simulink model "mrefrobotarm_modified_previous_y_previous_u_previous_ref"  (R2018b)
settings: Solver=FixedStepAuto  StartTime=0.0  StopTime=10  RelTol=1e-3  AbsTol=1e-6
undefined symbols (not defined in the file or in its folder): options, sfunxy2
libraries: neural x949, simulink x1
(part 17 of 31)

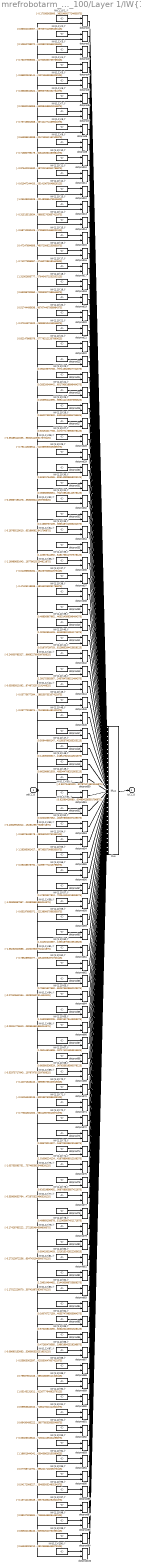
== system mrefrobotarm_modified_previous_y_previous_u_previous_ref/const_51traces_100/Layer 1/IW{1,1} ==
  "pd{1,1}" : Inport  PortDimensions=10
      mask Display: e = 0.06;c1 = [120 230 180]/255;c2 = ([120 230 180]+0)/(256+128);c3 = ([120 230 180]+128)/(256+128);patch([0 1 1 0],[0 0 1 1],c1);patch([0 1 1 1-e 1-e 0+e],[0 0 1 1-e 0+e 0+e],c2);patch([0 0 1 1-e 0+e 0+e],[0 1 1 1-e 1-e 0+e],c3);plot([0 1 1 0 0],[0 0 1 1 0]);
  "IW{1,1}(1,:)'" : Constant  Value=[-0.170305638008138859884610383232939057052135467529296875;-0.84091694602573696659675306364079006016254425048828125;-1.0473111215097110626714993486530147492885589599609375;-0.75666745499568965893644190146005712449550628662109375;0.1371939523011656281159531545199570246040821075439453125;-0.2076176579548360268123730065781273879110813140869140625;0.6369796280798090126751276329741813242435455322265625;0.9908763324366562930123336627730168402194976806640625;1.002178449147427041765467947698198258876800537109375;-0.82460061242790094748755791442818008363246917724609375]
      mask Display: e = 0.06;c1 = [120 150 230]/255;c2 = ([120 150 230]+0)/383;c3 = ([120 150 230]+128)/383;patch([0 1 1 0],[0 0 1 1],c1);patch([0 1 1 1-e 1-e 0+e],[0 0 1 1-e 0+e 0+e],c2);patch([0 0 1 1-e 0+e 0+e],[0 1 1 1-e 1-e 0+e],c3);plot([0 1 1 0 0],[0 0 1 1 0]);disp('Weights');
  "IW{1,1}(10,:)'" : Constant  Value=[-0.7188079917996403889191014968673698604106903076171875;-0.5527934950988353524081730938632972538471221923828125;1.177940059427081909149137572967447340488433837890625;-0.7566037792006319318005580498720519244670867919921875;0.10224905637283122905589749507271335460245609283447265625;0.880612868538781068394882822758518159389495849609375;0.05599996081731146990723146927848574705421924591064453125;-0.5350580343929980386974420980550348758697509765625;-0.73962591974704261499340418595238588750362396240234375;-0.01401764490016039164943517647543558268807828426361083984375]
      mask Display: e = 0.06;c1 = [120 150 230]/255;c2 = ([120 150 230]+0)/383;c3 = ([120 150 230]+128)/383;patch([0 1 1 0],[0 0 1 1],c1);patch([0 1 1 1-e 1-e 0+e],[0 0 1 1-e 0+e 0+e],c2);patch([0 0 1 1-e 0+e 0+e],[0 1 1 1-e 1-e 0+e],c3);plot([0 1 1 0 0],[0 0 1 1 0]);disp('Weights');
  "IW{1,1}(100,:)'" : Constant  Value=[0.64533025212050676433506168905296362936496734619140625;0.8803140978111179126841534525738097727298736572265625;0.54439970602968112967090519305202178657054901123046875;-0.53792355137469483050693952463916502892971038818359375;-1.2233752874797414467167300244909711182117462158203125;-0.375810009441459980106259308740845881402492523193359375;0.40564792046065389907738563124439679086208343505859375;0.542278062316380538021576285245828330516815185546875;0.338638468446645746201539850517292506992816925048828125;-0.05135870021747131197731306428977404721081256866455078125]
      mask Display: e = 0.06;c1 = [120 150 230]/255;c2 = ([120 150 230]+0)/383;c3 = ([120 150 230]+128)/383;patch([0 1 1 0],[0 0 1 1],c1);patch([0 1 1 1-e 1-e 0+e],[0 0 1 1-e 0+e 0+e],c2);patch([0 0 1 1-e 0+e 0+e],[0 1 1 1-e 1-e 0+e],c3);plot([0 1 1 0 0],[0 0 1 1 0]);disp('Weights');
  "IW{1,1}(11,:)'" : Constant  Value=[-0.97642024630729606915480189854861237108707427978515625;0.66445209408851069188273186227888800203800201416015625;-0.8919160165742419099643711888347752392292022705078125;0.10756129521181546915276072695633047260344028472900390625;-0.6447824446878331894339453356224112212657928466796875;0.67602283036553612038943583684158511459827423095703125;1.0285614969354053283012717656674794852733612060546875;-0.77894280059782949887647873765672557055950164794921875;-0.1748333285319037810889852835316560231149196624755859375;-0.41474870595583002153006191292661242187023162841796875]
      mask Display: e = 0.06;c1 = [120 150 230]/255;c2 = ([120 150 230]+0)/383;c3 = ([120 150 230]+128)/383;patch([0 1 1 0],[0 0 1 1],c1);patch([0 1 1 1-e 1-e 0+e],[0 0 1 1-e 0+e 0+e],c2);patch([0 0 1 1-e 0+e 0+e],[0 1 1 1-e 1-e 0+e],c3);plot([0 1 1 0 0],[0 0 1 1 0]);disp('Weights');
  "IW{1,1}(12,:)'" : Constant  Value=[-0.6194724442048145096606504012015648186206817626953125;-0.72861833503561956870697713384288363158702850341796875;1.103333456587284100436363587505184113979339599609375;-0.70243798980666405373796123967622406780719757080078125;0.439153999977970499468682419319520704448223114013671875;0.45345915572852302233286536647938191890716552734375;-0.34918842111248615811547324483399279415607452392578125;-0.8964166863968896503678251974633894860744476318359375;-0.43450253988920584102828570394194684922695159912109375;0.1004094661472918759148598155661602504551410675048828125]
      mask Display: e = 0.06;c1 = [120 150 230]/255;c2 = ([120 150 230]+0)/383;c3 = ([120 150 230]+128)/383;patch([0 1 1 0],[0 0 1 1],c1);patch([0 1 1 1-e 1-e 0+e],[0 0 1 1-e 0+e 0+e],c2);patch([0 0 1 1-e 0+e 0+e],[0 1 1 1-e 1-e 0+e],c3);plot([0 1 1 0 0],[0 0 1 1 0]);disp('Weights');
  "IW{1,1}(13,:)'" : Constant  Value=[1.25349304526054883268670891993679106235504150390625;-0.278560517477228819505086221397505141794681549072265625;0.730108871976856477203909889794886112213134765625;-0.549904814972676181383803850621916353702545166015625;0.62399252602846766446731407995685003697872161865234375;-1.281837938187930792111046685022301971912384033203125;0.345251730969751757793773094817879609763622283935546875;0.138568870452370263013364137805183418095111846923828125;-0.58106563584299875113714506369433365762233734130859375;-0.36006533748797819871612091446877457201480865478515625]
      mask Display: e = 0.06;c1 = [120 150 230]/255;c2 = ([120 150 230]+0)/383;c3 = ([120 150 230]+128)/383;patch([0 1 1 0],[0 0 1 1],c1);patch([0 1 1 1-e 1-e 0+e],[0 0 1 1-e 0+e 0+e],c2);patch([0 0 1 1-e 0+e 0+e],[0 1 1 1-e 1-e 0+e],c3);plot([0 1 1 0 0],[0 0 1 1 0]);disp('Weights');
  "IW{1,1}(14,:)'" : Constant  Value=[-0.3151351363461738497306896533700637519359588623046875;-0.0097595836595271122371197947131804539822041988372802734375;1.10936805191082843435879112803377211093902587890625;-0.93905292104770021754944764325045980513095855712890625;-0.9138700935437042982556476999889127910137176513671875;0.18374239433762584727816147278645075857639312744140625;1.069462447122071946381538509740494191646575927734375;-0.81828312627598853712385107428417541086673736572265625;-0.023265579288859618289908581800773390568792819976806640625;0.1571687035658450859454404735515709035098552703857421875]
      mask Display: e = 0.06;c1 = [120 150 230]/255;c2 = ([120 150 230]+0)/383;c3 = ([120 150 230]+128)/383;patch([0 1 1 0],[0 0 1 1],c1);patch([0 1 1 1-e 1-e 0+e],[0 0 1 1-e 0+e 0+e],c2);patch([0 0 1 1-e 0+e 0+e],[0 1 1 1-e 1-e 0+e],c3);plot([0 1 1 0 0],[0 0 1 1 0]);disp('Weights');
  "IW{1,1}(15,:)'" : Constant  Value=[-0.5871293042540719486765965484664775431156158447265625;0.3940422689418039414732675140840001404285430908203125;0.96312911671125911450275225433870218694210052490234375;-1.01431590084022449360645623528398573398590087890625;-0.325931841206041406078242061994387768208980560302734375;0.200414918554812360174111063315649516880512237548828125;0.331194186191319073220284963099402375519275665283203125;1.2119257407114261138048050270299427211284637451171875;-0.8267099033237830241205301717855036258697509765625;0.10958005298265061089324490239960141479969024658203125]
      mask Display: e = 0.06;c1 = [120 150 230]/255;c2 = ([120 150 230]+0)/383;c3 = ([120 150 230]+128)/383;patch([0 1 1 0],[0 0 1 1],c1);patch([0 1 1 1-e 1-e 0+e],[0 0 1 1-e 0+e 0+e],c2);patch([0 0 1 1-e 0+e 0+e],[0 1 1 1-e 1-e 0+e],c3);plot([0 1 1 0 0],[0 0 1 1 0]);disp('Weights');
  "IW{1,1}(16,:)'" : Constant  Value=[0.472476948566088517100780563851003535091876983642578125;0.436399456262539231499175684803049080073833465576171875;1.0138022013108933805369815672747790813446044921875;-0.825843001599289916470070238574407994747161865234375;0.239318836898521347666957126421038992702960968017578125;-0.6405951194830503681032496388070285320281982421875;-0.71669483108157117090541987636242993175983428955078125;-0.5155833539305538781860605013207532465457916259765625;0.320021634560399836910704607362276874482631683349609375;1.1416495802142418991564909447333775460720062255859375]
      mask Display: e = 0.06;c1 = [120 150 230]/255;c2 = ([120 150 230]+0)/383;c3 = ([120 150 230]+128)/383;patch([0 1 1 0],[0 0 1 1],c1);patch([0 1 1 1-e 1-e 0+e],[0 0 1 1-e 0+e 0+e],c2);patch([0 0 1 1-e 0+e 0+e],[0 1 1 1-e 1-e 0+e],c3);plot([0 1 1 0 0],[0 0 1 1 0]);disp('Weights');
  "IW{1,1}(17,:)'" : Constant  Value=[-0.74077896967243128667490736916079185903072357177734375;-0.2975123869242335405971289219451136887073516845703125;0.39331342274744585107981720284442417323589324951171875;-0.12030082952774480420377045675195404328405857086181640625;0.97014414268526094620170852067531086504459381103515625;-0.8509573298599459878488460162770934402942657470703125;-0.82800102302075317961538303279667161405086517333984375;0.86967158602187566440733235140214674174785614013671875;-0.314482355644385702664322934651863761246204376220703125;0.42603053129348611438587113298126496374607086181640625]
      mask Display: e = 0.06;c1 = [120 150 230]/255;c2 = ([120 150 230]+0)/383;c3 = ([120 150 230]+128)/383;patch([0 1 1 0],[0 0 1 1],c1);patch([0 1 1 1-e 1-e 0+e],[0 0 1 1-e 0+e 0+e],c2);patch([0 0 1 1-e 0+e 0+e],[0 1 1 1-e 1-e 0+e],c3);plot([0 1 1 0 0],[0 0 1 1 0]);disp('Weights');
  "IW{1,1}(18,:)'" : Constant  Value=[1.3100269377766393663620192455709911882877349853515625;-0.57664102931916350058827447355724871158599853515625;0.326570474994216708441996388501138426363468170166015625;-0.307961676870106060288634353128145448863506317138671875;0.82859508544864846069089026059373281896114349365234375;1.160795476552283655991004707175306975841522216796875;-0.0156597094076652391947401810057272086851298809051513671875;-0.350765766554864522053236441934132017195224761962890625;-0.058250586835098878968342006601233151741325855255126953125;-0.81675852122060366156119926017709076404571533203125]
      mask Display: e = 0.06;c1 = [120 150 230]/255;c2 = ([120 150 230]+0)/383;c3 = ([120 150 230]+128)/383;patch([0 1 1 0],[0 0 1 1],c1);patch([0 1 1 1-e 1-e 0+e],[0 0 1 1-e 0+e 0+e],c2);patch([0 0 1 1-e 0+e 0+e],[0 1 1 1-e 1-e 0+e],c3);plot([0 1 1 0 0],[0 0 1 1 0]);disp('Weights');
  "IW{1,1}(19,:)'" : Constant  Value=[0.632867829608980247968474941444583237171173095703125;-0.0743945784967924572672615113333449698984622955322265625;-0.91327949984337830624525622624787501990795135498046875;-0.82963064081226456369932975576375611126422882080078125;0.46425932832785410386833291340735740959644317626953125;0.462075831172123641099602764370501972734928131103515625;-0.4812285572585504045406423756503500044345855712890625;-0.01180364781508570770629518165151239372789859771728515625;-1.21000651010020288111945774289779365062713623046875;-1.0575192814166551880106226235511712729930877685546875]
      mask Display: e = 0.06;c1 = [120 150 230]/255;c2 = ([120 150 230]+0)/383;c3 = ([120 150 230]+128)/383;patch([0 1 1 0],[0 0 1 1],c1);patch([0 1 1 1-e 1-e 0+e],[0 0 1 1-e 0+e 0+e],c2);patch([0 0 1 1-e 0+e 0+e],[0 1 1 1-e 1-e 0+e],c3);plot([0 1 1 0 0],[0 0 1 1 0]);disp('Weights');
  "IW{1,1}(2,:)'" : Constant  Value=[0.86302163357631755946641760601778514683246612548828125;-0.5579812505175449910410634402069263160228729248046875;-0.8557487905362055613522898056544363498687744140625;-0.514363216250348642688550171442329883575439453125;-0.975544136415781082405374036170542240142822265625;0.4210426174550914169003590359352529048919677734375;-0.63869385442526571683430347547982819378376007080078125;0.65062821069079068703189250300056301057338714599609375;0.35157843060015958602804175825440324842929840087890625;0.86647648865104731630282230980810709297657012939453125]
      mask Display: e = 0.06;c1 = [120 150 230]/255;c2 = ([120 150 230]+0)/383;c3 = ([120 150 230]+128)/383;patch([0 1 1 0],[0 0 1 1],c1);patch([0 1 1 1-e 1-e 0+e],[0 0 1 1-e 0+e 0+e],c2);patch([0 0 1 1-e 0+e 0+e],[0 1 1 1-e 1-e 0+e],c3);plot([0 1 1 0 0],[0 0 1 1 0]);disp('Weights');
  "IW{1,1}(20,:)'" : Constant  Value=[0.51744495636959675355370791294262744486331939697265625;-0.1547734165125060623591224384654196910560131072998046875;-0.99093210573097934013020449128816835582256317138671875;0.263933305768935422275234259359422139823436737060546875;-0.0728289172390254313516066986267105676233768463134765625;-0.47621939097836063492508174022077582776546478271484375;-1.1292248128611817037381115369498729705810546875;-0.041618293867331478119719889718908234499394893646240234375;-1.0841222482710100027958333157585002481937408447265625;0.189330866318472512688231290667317807674407958984375]
      mask Display: e = 0.06;c1 = [120 150 230]/255;c2 = ([120 150 230]+0)/383;c3 = ([120 150 230]+128)/383;patch([0 1 1 0],[0 0 1 1],c1);patch([0 1 1 1-e 1-e 0+e],[0 0 1 1-e 0+e 0+e],c2);patch([0 0 1 1-e 0+e 0+e],[0 1 1 1-e 1-e 0+e],c3);plot([0 1 1 0 0],[0 0 1 1 0]);disp('Weights');
  "IW{1,1}(21,:)'" : Constant  Value=[-0.371518715204130212104161046227090992033481597900390625;0.467337757155769306649517602636478841304779052734375;0.2269719081821011397170906320752692408859729766845703125;0.08481228167460937161781231452550855465233325958251953125;1.44458428183304032899059166084043681621551513671875;-0.0234380543474412873783396804583389894105494022369384765625;-0.45455741294511387007304392682272009551525115966796875;-1.227396331157477593620797051698900759220123291015625;1.004787797655553038822517919470556080341339111328125;0.1506891507751337566656246735874447040259838104248046875]
      mask Display: e = 0.06;c1 = [120 150 230]/255;c2 = ([120 150 230]+0)/383;c3 = ([120 150 230]+128)/383;patch([0 1 1 0],[0 0 1 1],c1);patch([0 1 1 1-e 1-e 0+e],[0 0 1 1-e 0+e 0+e],c2);patch([0 0 1 1-e 0+e 0+e],[0 1 1 1-e 1-e 0+e],c3);plot([0 1 1 0 0],[0 0 1 1 0]);disp('Weights');
  "IW{1,1}(22,:)'" : Constant  Value=[0.8214786607933863837871513169375248253345489501953125;-0.84220472360854403692798086922266520559787750244140625;-0.4880387325338571002930621034465730190277099609375;0.60696914376156396730976894104969687759876251220703125;-0.887166316198694016037507026339881122112274169921875;0.79926168947075215687192439872887916862964630126953125;0.80816360662084540944505306470091454684734344482421875;-0.5721497555960544101338882683194242417812347412109375;0.567110586128520832716048971633426845073699951171875;0.460100559308461110052945741699659265577793121337890625]
      mask Display: e = 0.06;c1 = [120 150 230]/255;c2 = ([120 150 230]+0)/383;c3 = ([120 150 230]+128)/383;patch([0 1 1 0],[0 0 1 1],c1);patch([0 1 1 1-e 1-e 0+e],[0 0 1 1-e 0+e 0+e],c2);patch([0 0 1 1-e 0+e 0+e],[0 1 1 1-e 1-e 0+e],c3);plot([0 1 1 0 0],[0 0 1 1 0]);disp('Weights');
  "IW{1,1}(23,:)'" : Constant  Value=[0.09419575738046971624672920597731717862188816070556640625;0.411730692981060186763642150253872387111186981201171875;0.41947599709186744743050212491652928292751312255859375;-0.51148504298385499833301537364604882895946502685546875;-0.70916810981691391635450827379827387630939483642578125;-1.16257670448549976782715020817704498767852783203125;-0.9791973104793552096225539571605622768402099609375;1.0943516112241928883719310761080123484134674072265625;0.3134970998681072540392733571934513747692108154296875;0.379077417386230075546649231910123489797115325927734375]
      mask Display: e = 0.06;c1 = [120 150 230]/255;c2 = ([120 150 230]+0)/383;c3 = ([120 150 230]+128)/383;patch([0 1 1 0],[0 0 1 1],c1);patch([0 1 1 1-e 1-e 0+e],[0 0 1 1-e 0+e 0+e],c2);patch([0 0 1 1-e 0+e 0+e],[0 1 1 1-e 1-e 0+e],c3);plot([0 1 1 0 0],[0 0 1 1 0]);disp('Weights');
  "IW{1,1}(24,:)'" : Constant  Value=[0.283200494423681170541584606326068751513957977294921875;-0.5446401217881791101405042354599572718143463134765625;-0.926718550507767968582584217074327170848846435546875;1.0023171860421360435111637343652546405792236328125;-0.401982680773332823331855934156919829547405242919921875;0.255525526075908226975030856920056976377964019775390625;0.89032793712451674394969813874922692775726318359375;1.0527621924029799682642760672024451196193695068359375;-0.36601162666097974973666850928566418588161468505859375;-0.6552325421269118432832101461826823651790618896484375]
      mask Display: e = 0.06;c1 = [120 150 230]/255;c2 = ([120 150 230]+0)/383;c3 = ([120 150 230]+128)/383;patch([0 1 1 0],[0 0 1 1],c1);patch([0 1 1 1-e 1-e 0+e],[0 0 1 1-e 0+e 0+e],c2);patch([0 0 1 1-e 0+e 0+e],[0 1 1 1-e 1-e 0+e],c3);plot([0 1 1 0 0],[0 0 1 1 0]);disp('Weights');
  "IW{1,1}(25,:)'" : Constant  Value=[0.263952423958710491458390379193588159978389739990234375;0.5179072584720512129052849559229798614978790283203125;-0.07410029705099137331547609619519789703190326690673828125;-0.871104755366767680158091025077737867832183837890625;-0.903016070580165308712139449198730289936065673828125;0.7666990005644398475936895920312963426113128662109375;-0.8009951831969763791363448035554029047489166259765625;0.2222925408359026910876110605386202223598957061767578125;0.925174136198293250998858638922683894634246826171875;-0.86957339748055384465175166042172349989414215087890625]
      mask Display: e = 0.06;c1 = [120 150 230]/255;c2 = ([120 150 230]+0)/383;c3 = ([120 150 230]+128)/383;patch([0 1 1 0],[0 0 1 1],c1);patch([0 1 1 1-e 1-e 0+e],[0 0 1 1-e 0+e 0+e],c2);patch([0 0 1 1-e 0+e 0+e],[0 1 1 1-e 1-e 0+e],c3);plot([0 1 1 0 0],[0 0 1 1 0]);disp('Weights');
  "IW{1,1}(26,:)'" : Constant  Value=[0.66207392930839847888790927754598669707775115966796875;-0.927826293094271559169783358811400830745697021484375;-0.53992479788772340665303772766492329537868499755859375;0.6093454934288307089929048743215389549732208251953125;-0.935697886848097848400129805668257176876068115234375;0.1275534011237173526165378234509262256324291229248046875;-0.71002476471670294966287428906070999801158905029296875;-0.6154051848111132816399049261235632002353668212890625;1.1040911523030134677725300207384862005710601806640625;-0.006260111974622986109884070771158803836442530155181884765625]
      mask Display: e = 0.06;c1 = [120 150 230]/255;c2 = ([120 150 230]+0)/383;c3 = ([120 150 230]+128)/383;patch([0 1 1 0],[0 0 1 1],c1);patch([0 1 1 1-e 1-e 0+e],[0 0 1 1-e 0+e 0+e],c2);patch([0 0 1 1-e 0+e 0+e],[0 1 1 1-e 1-e 0+e],c3);plot([0 1 1 0 0],[0 0 1 1 0]);disp('Weights');
  "IW{1,1}(27,:)'" : Constant  Value=[0.6319401773805248812010404435568489134311676025390625;-0.84957682223790575992694584783748723566532135009765625;0.5357136767300738622310518621816299855709075927734375;-0.88565078629698656964563951987656764686107635498046875;-1.0552096523122538318517626976245082914829254150390625;0.88306545275100223335584814776666462421417236328125;0.826385453474836051412921733572147786617279052734375;0.046199217615886183085915916990416008047759532928466796875;-0.2139731479252826584769309192779473960399627685546875;0.07682384842362673105231607451059971936047077178955078125]
      mask Display: e = 0.06;c1 = [120 150 230]/255;c2 = ([120 150 230]+0)/383;c3 = ([120 150 230]+128)/383;patch([0 1 1 0],[0 0 1 1],c1);patch([0 1 1 1-e 1-e 0+e],[0 0 1 1-e 0+e 0+e],c2);patch([0 0 1 1-e 0+e 0+e],[0 1 1 1-e 1-e 0+e],c3);plot([0 1 1 0 0],[0 0 1 1 0]);disp('Weights');
  "IW{1,1}(28,:)'" : Constant  Value=[-0.39489441535742753064397447815281338989734649658203125;0.047164668367843463891997402015476836822926998138427734375;0.73428078885034953060539919533766806125640869140625;-0.5170768242902992195553224519244395196437835693359375;-0.650913494200199949091256712563335895538330078125;-0.29069613486833978388546029236749745905399322509765625;0.685236331361608108636573888361454010009765625;1.4916971807746828293517182828509248793125152587890625;0.8581651008094379751156566271674819290637969970703125;-0.0231304909361202577777749667120588128454983234405517578125]
      mask Display: e = 0.06;c1 = [120 150 230]/255;c2 = ([120 150 230]+0)/383;c3 = ([120 150 230]+128)/383;patch([0 1 1 0],[0 0 1 1],c1);patch([0 1 1 1-e 1-e 0+e],[0 0 1 1-e 0+e 0+e],c2);patch([0 0 1 1-e 0+e 0+e],[0 1 1 1-e 1-e 0+e],c3);plot([0 1 1 0 0],[0 0 1 1 0]);disp('Weights');
  "IW{1,1}(29,:)'" : Constant  Value=[-0.791116069143575462163653355673886835575103759765625;-0.5164163335247102804004271092708222568035125732421875;1.134330783552872201624950321274809539318084716796875;-0.50120208438853131038825949872261844575405120849609375;1.31633127280354500499015557579696178436279296875;-0.266539812518394481077876889685285277664661407470703125;-1.1946739896386346924117560774902813136577606201171875;-0.87808470016394990498298511738539673388004302978515625;0.55821663455198378134269887596019543707370758056640625;-0.49625539141540497833915424052975140511989593505859375]
      mask Display: e = 0.06;c1 = [120 150 230]/255;c2 = ([120 150 230]+0)/383;c3 = ([120 150 230]+128)/383;patch([0 1 1 0],[0 0 1 1],c1);patch([0 1 1 1-e 1-e 0+e],[0 0 1 1-e 0+e 0+e],c2);patch([0 0 1 1-e 0+e 0+e],[0 1 1 1-e 1-e 0+e],c3);plot([0 1 1 0 0],[0 0 1 1 0]);disp('Weights');
  "IW{1,1}(3,:)'" : Constant  Value=[0.10552788972297309777470530889331712387502193450927734375;0.88774397676408056678809543882380239665508270263671875;-0.290424624436791900539134303471655584871768951416015625;-0.55515280106611630817070590637740679085254669189453125;0.2495591789322011144758306500079925172030925750732421875;0.518666085829210476987327638198621571063995361328125;-0.7146768557075773298237209019134752452373504638671875;-1.1663537558078445055542715635965578258037567138671875;-0.8429764640291583788211937644518911838531494140625;-0.9813004957389550586555060363025404512882232666015625]
      mask Display: e = 0.06;c1 = [120 150 230]/255;c2 = ([120 150 230]+0)/383;c3 = ([120 150 230]+128)/383;patch([0 1 1 0],[0 0 1 1],c1);patch([0 1 1 1-e 1-e 0+e],[0 0 1 1-e 0+e 0+e],c2);patch([0 0 1 1-e 0+e 0+e],[0 1 1 1-e 1-e 0+e],c3);plot([0 1 1 0 0],[0 0 1 1 0]);disp('Weights');
  "IW{1,1}(30,:)'" : Constant  Value=[0.626017640653714568799159678746946156024932861328125;0.1479782944948506429039269960412639193236827850341796875;0.1393829123997244734400879906388581730425357818603515625;-0.466620041588095502138600068064988590776920318603515625;0.66086884231012976709251915963250212371349334716796875;-0.471986669595617691630451417950098402798175811767578125;-0.2210552926631040027150021387569722719490528106689453125;-1.1080786045275470286242125439457595348358154296875;0.834856584082876107544279875583015382289886474609375;-1.1414665398944816576687344422680325806140899658203125]
      mask Display: e = 0.06;c1 = [120 150 230]/255;c2 = ([120 150 230]+0)/383;c3 = ([120 150 230]+128)/383;patch([0 1 1 0],[0 0 1 1],c1);patch([0 1 1 1-e 1-e 0+e],[0 0 1 1-e 0+e 0+e],c2);patch([0 0 1 1-e 0+e 0+e],[0 1 1 1-e 1-e 0+e],c3);plot([0 1 1 0 0],[0 0 1 1 0]);disp('Weights');
  "IW{1,1}(31,:)'" : Constant  Value=[0.06668568061349466891130077783600427210330963134765625;0.88698937972517466477029302041046321392059326171875;-0.5020620907164901058905570607748813927173614501953125;0.187274332582882896414133711004978977143764495849609375;0.88575747583989616895649987782235257327556610107421875;-0.81825415593434147609741557971574366092681884765625;0.68899848459867774064235845798975788056850433349609375;0.94305114029854142376763093125191517174243927001953125;-0.6691163549777299213161541047156788408756256103515625;0.0737283603405594067936590363387949764728546142578125]
      mask Display: e = 0.06;c1 = [120 150 230]/255;c2 = ([120 150 230]+0)/383;c3 = ([120 150 230]+128)/383;patch([0 1 1 0],[0 0 1 1],c1);patch([0 1 1 1-e 1-e 0+e],[0 0 1 1-e 0+e 0+e],c2);patch([0 0 1 1-e 0+e 0+e],[0 1 1 1-e 1-e 0+e],c3);plot([0 1 1 0 0],[0 0 1 1 0]);disp('Weights');
  "IW{1,1}(32,:)'" : Constant  Value=[-0.29867193478553277774523166954168118536472320556640625;1.060980638567496026070102743688039481639862060546875;-0.83983801109680944474433772484189830720424652099609375;0.287629578909353422755401652466389350593090057373046875;0.51783125481217850971660254799644462764263153076171875;0.283346881376406456443106662845821119844913482666015625;-0.9786366480410244594878577117924578487873077392578125;-1.067149516731294323079737296211533248424530029296875;0.2003698181893468766023858051994466222822666168212890625;-0.67592741568701220078452251982525922358036041259765625]
      mask Display: e = 0.06;c1 = [120 150 230]/255;c2 = ([120 150 230]+0)/383;c3 = ([120 150 230]+128)/383;patch([0 1 1 0],[0 0 1 1],c1);patch([0 1 1 1-e 1-e 0+e],[0 0 1 1-e 0+e 0+e],c2);patch([0 0 1 1-e 0+e 0+e],[0 1 1 1-e 1-e 0+e],c3);plot([0 1 1 0 0],[0 0 1 1 0]);disp('Weights');
  "IW{1,1}(33,:)'" : Constant  Value=[0.116887874095150390285624553143861703574657440185546875;0.63308229908039714839418365954770706593990325927734375;-0.0777111172460257793037641249611624516546726226806640625;-0.78538148508143701409522918766015209257602691650390625;-0.99080372460652810229220222026924602687358856201171875;1.1750499935507499049691659820382483303546905517578125;-0.50299687336723286623652029447839595377445220947265625;-0.2186709169920443007750776587272412143647670745849609375;1.1043639607425597137790873603080399334430694580078125;-0.33939116012177217296397202517255209386348724365234375]
      mask Display: e = 0.06;c1 = [120 150 230]/255;c2 = ([120 150 230]+0)/383;c3 = ([120 150 230]+128)/383;patch([0 1 1 0],[0 0 1 1],c1);patch([0 1 1 1-e 1-e 0+e],[0 0 1 1-e 0+e 0+e],c2);patch([0 0 1 1-e 0+e 0+e],[0 1 1 1-e 1-e 0+e],c3);plot([0 1 1 0 0],[0 0 1 1 0]);disp('Weights');
  "IW{1,1}(34,:)'" : Constant  Value=[-0.187692190106364675816763565308065153658390045166015625;1.2964434572948750901133507795748300850391387939453125;-0.46176563770852829815538598268176428973674774169921875;-0.27552557411780764784481334572774358093738555908203125;-0.603843694195803859514626310556195676326751708984375;-0.5983048122454321937624399652122519910335540771484375;-0.7669376889578789491253019150462932884693145751953125;0.1629662413332511883279352105091675184667110443115234375;0.324312279636630729218182978002005256712436676025390625;-0.20198865888583827921110014358418993651866912841796875]
      mask Display: e = 0.06;c1 = [120 150 230]/255;c2 = ([120 150 230]+0)/383;c3 = ([120 150 230]+128)/383;patch([0 1 1 0],[0 0 1 1],c1);patch([0 1 1 1-e 1-e 0+e],[0 0 1 1-e 0+e 0+e],c2);patch([0 0 1 1-e 0+e 0+e],[0 1 1 1-e 1-e 0+e],c3);plot([0 1 1 0 0],[0 0 1 1 0]);disp('Weights');
  "IW{1,1}(35,:)'" : Constant  Value=[1.2256734439276437687027510037296451628208160400390625;-0.9330947970269434232903904558042995631694793701171875;0.131230327499476773223108239108114503324031829833984375;-0.6805497732182999026662173491786234080791473388671875;0.62001055341251010144532074264134280383586883544921875;0.6535912239619818819846841506659984588623046875;0.62055220915618836130533964023925364017486572265625;0.358587438438109640248541154505801387131214141845703125;-0.61424990739872475931093731560395099222660064697265625;-0.6624892400696531513659692791406996548175811767578125]
      mask Display: e = 0.06;c1 = [120 150 230]/255;c2 = ([120 150 230]+0)/383;c3 = ([120 150 230]+128)/383;patch([0 1 1 0],[0 0 1 1],c1);patch([0 1 1 1-e 1-e 0+e],[0 0 1 1-e 0+e 0+e],c2);patch([0 0 1 1-e 0+e 0+e],[0 1 1 1-e 1-e 0+e],c3);plot([0 1 1 0 0],[0 0 1 1 0]);disp('Weights');
  "IW{1,1}(36,:)'" : Constant  Value=[-1.1698983164396683509522745225694961845874786376953125;0.039703620286117603799258546359851607121527194976806640625;0.07486672289221334153364040275846491567790508270263671875;0.9785601315053107374097862702910788357257843017578125;0.980185417500065714335732991457916796207427978515625;-0.66657049432687376366857279208488762378692626953125;0.5239409712108564765031815113616175949573516845703125;-0.2496624487829249561254840727997361682355403900146484375;-0.86867630952089813778371762964525260031223297119140625;-0.370817217133690923969169261908973567187786102294921875]
      mask Display: e = 0.06;c1 = [120 150 230]/255;c2 = ([120 150 230]+0)/383;c3 = ([120 150 230]+128)/383;patch([0 1 1 0],[0 0 1 1],c1);patch([0 1 1 1-e 1-e 0+e],[0 0 1 1-e 0+e 0+e],c2);patch([0 0 1 1-e 0+e 0+e],[0 1 1 1-e 1-e 0+e],c3);plot([0 1 1 0 0],[0 0 1 1 0]);disp('Weights');
  "IW{1,1}(37,:)'" : Constant  Value=[-0.0149666328452099338386371840670108213089406490325927734375;-0.931936877760145332416641394956968724727630615234375;-1.151949433050794002753036693320609629154205322265625;0.86870508548147118421667300935951061546802520751953125;0.187403977636498686454302742276922799646854400634765625;1.008057905890814343052852564142085611820220947265625;0.092644828769221698738789427807205356657505035400390625;-0.73461588425985924200034560271888040006160736083984375;0.5612002737993935230775832678773440420627593994140625;-0.10958425546422807805857502216895227320492267608642578125]
      mask Display: e = 0.06;c1 = [120 150 230]/255;c2 = ([120 150 230]+0)/383;c3 = ([120 150 230]+128)/383;patch([0 1 1 0],[0 0 1 1],c1);patch([0 1 1 1-e 1-e 0+e],[0 0 1 1-e 0+e 0+e],c2);patch([0 0 1 1-e 0+e 0+e],[0 1 1 1-e 1-e 0+e],c3);plot([0 1 1 0 0],[0 0 1 1 0]);disp('Weights');
  "IW{1,1}(38,:)'" : Constant  Value=[-0.474251185983347089969441867651767097413539886474609375;0.66920382643324760607583812088705599308013916015625;0.64710109619507372169522341209813021123409271240234375;-0.51139914103564210190455696647404693067073822021484375;-0.63816283216853098014809120286372490227222442626953125;0.29697077566583074403894215720356442034244537353515625;-0.71411559907816102299449312340584583580493927001953125;-0.340996826896414029217652341685607098042964935302734375;-1.3192546636798339054763573585660196840763092041015625;-0.83402969627138634489682544881361536681652069091796875]
      mask Display: e = 0.06;c1 = [120 150 230]/255;c2 = ([120 150 230]+0)/383;c3 = ([120 150 230]+128)/383;patch([0 1 1 0],[0 0 1 1],c1);patch([0 1 1 1-e 1-e 0+e],[0 0 1 1-e 0+e 0+e],c2);patch([0 0 1 1-e 0+e 0+e],[0 1 1 1-e 1-e 0+e],c3);plot([0 1 1 0 0],[0 0 1 1 0]);disp('Weights');
  "IW{1,1}(39,:)'" : Constant  Value=[0.4885696796264940022780365325161255896091461181640625;1.0011953446721630900384525375557132065296173095703125;-0.07965199188943576646959598974717664532363414764404296875;-0.14133535981193434682978704586275853216648101806640625;0.7405218790532515082958298080484382808208465576171875;-0.08748518407597898061123231627789209596812725067138671875;-0.13676008771209080538966418316704221069812774658203125;-0.97328788404739630113482462547835893929004669189453125;1.4107007557266684205643514360417611896991729736328125;0.035579408801526289651828705018488108180463314056396484375]
      mask Display: e = 0.06;c1 = [120 150 230]/255;c2 = ([120 150 230]+0)/383;c3 = ([120 150 230]+128)/383;patch([0 1 1 0],[0 0 1 1],c1);patch([0 1 1 1-e 1-e 0+e],[0 0 1 1-e 0+e 0+e],c2);patch([0 0 1 1-e 0+e 0+e],[0 1 1 1-e 1-e 0+e],c3);plot([0 1 1 0 0],[0 0 1 1 0]);disp('Weights');
  "IW{1,1}(4,:)'" : Constant  Value=[-0.76197969360801354188339473694213666021823883056640625;-0.26771973179288444111278977288748137652873992919921875;0.697379882929172634220549298333935439586639404296875;0.1355540479345000992594805211410857737064361572265625;0.52410901792617270444907262572087347507476806640625;-1.0158318151387122352247160961269401013851165771484375;0.8255710489851839639641184476204216480255126953125;-0.99875358677146852670603038859553635120391845703125;-0.71022033136298012845344373999978415668010711669921875;-0.706952677093088510673624114133417606353759765625]
      mask Display: e = 0.06;c1 = [120 150 230]/255;c2 = ([120 150 230]+0)/383;c3 = ([120 150 230]+128)/383;patch([0 1 1 0],[0 0 1 1],c1);patch([0 1 1 1-e 1-e 0+e],[0 0 1 1-e 0+e 0+e],c2);patch([0 0 1 1-e 0+e 0+e],[0 1 1 1-e 1-e 0+e],c3);plot([0 1 1 0 0],[0 0 1 1 0]);disp('Weights');
  "IW{1,1}(40,:)'" : Constant  Value=[1.022626944269706683598997187800705432891845703125;0.09685762306828386847268319570503081195056438446044921875;-0.64434950537638535639217707284842617809772491455078125;0.658483519736270839217695538536645472049713134765625;0.2395668410857852703710335617870441637933254241943359375;0.07937716463412373968377977462296257726848125457763671875;-1.009659204805799515014541611890308558940887451171875;1.149825552452031995898096283781342208385467529296875;-0.456427362312665729771055111996247433125972747802734375;0.52825004028654276577725568131427280604839324951171875]
      mask Display: e = 0.06;c1 = [120 150 230]/255;c2 = ([120 150 230]+0)/383;c3 = ([120 150 230]+128)/383;patch([0 1 1 0],[0 0 1 1],c1);patch([0 1 1 1-e 1-e 0+e],[0 0 1 1-e 0+e 0+e],c2);patch([0 0 1 1-e 0+e 0+e],[0 1 1 1-e 1-e 0+e],c3);plot([0 1 1 0 0],[0 0 1 1 0]);disp('Weights');
  "IW{1,1}(41,:)'" : Constant  Value=[0.0197973970311624315743248558874256559647619724273681640625;1.085813860034017697131503155105747282505035400390625;0.31872277303724427799380691794794984161853790283203125;-0.337555590416401984921179746379493735730648040771484375;-0.2287653370871609859182882473760400898754596710205078125;-1.15213675126067727205736446194350719451904296875;-1.072795236423661702218623759108595550060272216796875;-0.86041713033244204833493995465687476098537445068359375;0.2491044385743285960455040140004712156951427459716796875;0.0311716484729678451615075829295165021903812885284423828125]
      mask Display: e = 0.06;c1 = [120 150 230]/255;c2 = ([120 150 230]+0)/383;c3 = ([120 150 230]+128)/383;patch([0 1 1 0],[0 0 1 1],c1);patch([0 1 1 1-e 1-e 0+e],[0 0 1 1-e 0+e 0+e],c2);patch([0 0 1 1-e 0+e 0+e],[0 1 1 1-e 1-e 0+e],c3);plot([0 1 1 0 0],[0 0 1 1 0]);disp('Weights');
  "IW{1,1}(42,:)'" : Constant  Value=[-0.245097853277515820291654335960629396140575408935546875;-0.830880328293551517759851776645518839359283447265625;-0.2269993300405658553930976495394133962690830230712890625;0.829460478517292099098767721443437039852142333984375;1.0593027281025939601022400893270969390869140625;-0.402883002674919332708469710269127972424030303955078125;-1.40303812782332215647329576313495635986328125;0.2428443170749092494542509257371420972049236297607421875;-0.5168063761117320797922047859174199402332305908203125;-0.06895590557082743876637920266148285008966922760009765625]
      mask Display: e = 0.06;c1 = [120 150 230]/255;c2 = ([120 150 230]+0)/383;c3 = ([120 150 230]+128)/383;patch([0 1 1 0],[0 0 1 1],c1);patch([0 1 1 1-e 1-e 0+e],[0 0 1 1-e 0+e 0+e],c2);patch([0 0 1 1-e 0+e 0+e],[0 1 1 1-e 1-e 0+e],c3);plot([0 1 1 0 0],[0 0 1 1 0]);disp('Weights');
  "IW{1,1}(43,:)'" : Constant  Value=[1.39175382067646591366383290733210742473602294921875;-1.1139510165497885640917274940875358879566192626953125;0.1032497213740615482624463083993759937584400177001953125;-0.73879464515659964973792739328928291797637939453125;0.11409115966016024346085799834327190183103084564208984375;-0.88923187320735352923151140203117392957210540771484375;-0.1643381852559737954511120960887637920677661895751953125;-0.073600629219999602614876721418113447725772857666015625;0.458300780037487920370864458163850940763950347900390625;-0.15656873365645951334812480126856826245784759521484375]
      mask Display: e = 0.06;c1 = [120 150 230]/255;c2 = ([120 150 230]+0)/383;c3 = ([120 150 230]+128)/383;patch([0 1 1 0],[0 0 1 1],c1);patch([0 1 1 1-e 1-e 0+e],[0 0 1 1-e 0+e 0+e],c2);patch([0 0 1 1-e 0+e 0+e],[0 1 1 1-e 1-e 0+e],c3);plot([0 1 1 0 0],[0 0 1 1 0]);disp('Weights');
  "IW{1,1}(44,:)'" : Constant  Value=[-0.05565811092998625142502788776255329139530658721923828125;0.988680095798270652807104852399788796901702880859375;-0.330089164651135968941986220670514740049839019775390625;-0.86236260879891091235549538396298885345458984375;-0.423405769440457213637074573853169567883014678955078125;-0.301966554618198046444632609563996084034442901611328125;-1.0620394019968391052799461249378509819507598876953125;-0.6384245393665708423469595800270326435565948486328125;-0.174946884322957074697768575788359157741069793701171875;1.0292807807961354971126866075792349874973297119140625]
      mask Display: e = 0.06;c1 = [120 150 230]/255;c2 = ([120 150 230]+0)/383;c3 = ([120 150 230]+128)/383;patch([0 1 1 0],[0 0 1 1],c1);patch([0 1 1 1-e 1-e 0+e],[0 0 1 1-e 0+e 0+e],c2);patch([0 0 1 1-e 0+e 0+e],[0 1 1 1-e 1-e 0+e],c3);plot([0 1 1 0 0],[0 0 1 1 0]);disp('Weights');
  "IW{1,1}(45,:)'" : Constant  Value=[-0.037756773940375652764966929453294142149388790130615234375;1.1371216229658631657883915977436117827892303466796875;0.6667902293500593824404631959623657166957855224609375;-0.3108486294488315149209256560425274074077606201171875;-0.87481248056356297748692441018647514283657073974609375;0.456574357411410225449088784444029442965984344482421875;-1.3429313133410258895850120097748003900051116943359375;-0.42776873968760364963515030467533506453037261962890625;0.30455329901415895132998912231414578855037689208984375;0.1743134554016778359208927895451779477298259735107421875]
      mask Display: e = 0.06;c1 = [120 150 230]/255;c2 = ([120 150 230]+0)/383;c3 = ([120 150 230]+128)/383;patch([0 1 1 0],[0 0 1 1],c1);patch([0 1 1 1-e 1-e 0+e],[0 0 1 1-e 0+e 0+e],c2);patch([0 0 1 1-e 0+e 0+e],[0 1 1 1-e 1-e 0+e],c3);plot([0 1 1 0 0],[0 0 1 1 0]);disp('Weights');
  "IW{1,1}(46,:)'" : Constant  Value=[-0.037779198741022944341150235914028598926961421966552734375;1.120399950416423262566922858241014182567596435546875;-0.2136276573328312611277368660012143664062023162841796875;0.1214309664592614634859302213953924365341663360595703125;0.5924194879976327765547239323495887219905853271484375;-1.3620432198545753266216706833802163600921630859375;0.283133725670500047133515408859238959848880767822265625;-0.259000087925692124013465900134178809821605682373046875;-0.83319174909974547116320309214643202722072601318359375;-0.76470705793156745766481208192999474704265594482421875]
      mask Display: e = 0.06;c1 = [120 150 230]/255;c2 = ([120 150 230]+0)/383;c3 = ([120 150 230]+128)/383;patch([0 1 1 0],[0 0 1 1],c1);patch([0 1 1 1-e 1-e 0+e],[0 0 1 1-e 0+e 0+e],c2);patch([0 0 1 1-e 0+e 0+e],[0 1 1 1-e 1-e 0+e],c3);plot([0 1 1 0 0],[0 0 1 1 0]);disp('Weights');
  "IW{1,1}(47,:)'" : Constant  Value=[0.5094496014733189692691439631744287908077239990234375;0.217653922431265300918568073029746301472187042236328125;-0.92740217234425748049631010871962644159793853759765625;0.000386905548955825888228499120913284059497527778148651123046875;-0.89098275147228755965755908619030378758907318115234375;0.259615976810294968313286290140240453183650970458984375;-0.01182512539577553790925978915993255213834345340728759765625;0.4488253752788733397238729594391770660877227783203125;-1.0174566684678847394707190687768161296844482421875;-1.17159537776484246052177695673890411853790283203125]
      mask Display: e = 0.06;c1 = [120 150 230]/255;c2 = ([120 150 230]+0)/383;c3 = ([120 150 230]+128)/383;patch([0 1 1 0],[0 0 1 1],c1);patch([0 1 1 1-e 1-e 0+e],[0 0 1 1-e 0+e 0+e],c2);patch([0 0 1 1-e 0+e 0+e],[0 1 1 1-e 1-e 0+e],c3);plot([0 1 1 0 0],[0 0 1 1 0]);disp('Weights');
  "IW{1,1}(48,:)'" : Constant  Value=[0.143050365177295246699173958404571749269962310791015625;1.497275644643541792078167418367229402065277099609375;0.65999257750992035287396220155642367899417877197265625;1.16850303836929025891322453389875590801239013671875;-0.1467929645374324298945367672786233015358448028564453125;-0.31471114236739528013941935569164343178272247314453125;0.87888553239383038206966602956526912748813629150390625;-0.003192449795369928754185107067087301402352750301361083984375;0.28996208759709907187840371989295817911624908447265625;0.598644686846575790895030877436511218547821044921875]
      mask Display: e = 0.06;c1 = [120 150 230]/255;c2 = ([120 150 230]+0)/383;c3 = ([120 150 230]+128)/383;patch([0 1 1 0],[0 0 1 1],c1);patch([0 1 1 1-e 1-e 0+e],[0 0 1 1-e 0+e 0+e],c2);patch([0 0 1 1-e 0+e 0+e],[0 1 1 1-e 1-e 0+e],c3);plot([0 1 1 0 0],[0 0 1 1 0]);disp('Weights');
  "IW{1,1}(49,:)'" : Constant  Value=[0.66298961303626458008153576884069480001926422119140625;-0.82085278956611318346148209457169286906719207763671875;-0.70401651252550434545440793954185210168361663818359375;-0.97150427319233012557475603898637928068637847900390625;0.250234347062193218658165960732731036841869354248046875;0.81804110715012356980224694780190475285053253173828125;-0.43784860562585825594084099066094495356082916259765625;0.64248688031045819712971933768130838871002197265625;0.324631359683427100915054097640677355229854583740234375;0.855399134758077384077523674932308495044708251953125]
      mask Display: e = 0.06;c1 = [120 150 230]/255;c2 = ([120 150 230]+0)/383;c3 = ([120 150 230]+128)/383;patch([0 1 1 0],[0 0 1 1],c1);patch([0 1 1 1-e 1-e 0+e],[0 0 1 1-e 0+e 0+e],c2);patch([0 0 1 1-e 0+e 0+e],[0 1 1 1-e 1-e 0+e],c3);plot([0 1 1 0 0],[0 0 1 1 0]);disp('Weights');
  "IW{1,1}(5,:)'" : Constant  Value=[-0.8680252614191588111935971028287895023822784423828125;-0.09484493695201452745369152808052604086697101593017578125;0.70796218709212743736003403682843782007694244384765625;-0.98135506661690563579014678907697089016437530517578125;-0.75788320402631292882489333351259119808673858642578125;-0.329742848881782901759862625112873502075672149658203125;0.62704759100485230050026075332425534725189208984375;0.88132821955488349630059019546024501323699951171875;-0.24027900517276201686200920448754914104938507080078125;-0.80655538630496892427146349291433580219745635986328125]
      mask Display: e = 0.06;c1 = [120 150 230]/255;c2 = ([120 150 230]+0)/383;c3 = ([120 150 230]+128)/383;patch([0 1 1 0],[0 0 1 1],c1);patch([0 1 1 1-e 1-e 0+e],[0 0 1 1-e 0+e 0+e],c2);patch([0 0 1 1-e 0+e 0+e],[0 1 1 1-e 1-e 0+e],c3);plot([0 1 1 0 0],[0 0 1 1 0]);disp('Weights');
  "IW{1,1}(50,:)'" : Constant  Value=[-0.93275460320902248145813473456655628979206085205078125;-0.98162007550159791069432912991032935678958892822265625;-1.052484303446560520711727804155088961124420166015625;0.2280554726064465409507420190493576228618621826171875;0.53718835381505181114647484719171188771724700927734375;-0.88887188824303720036112963498453609645366668701171875;-0.63739942661443194094061936993966810405254364013671875;-0.51446719717050248821266222876147367060184478759765625;0.74085906660168709958469435150618664920330047607421875;0.393010406648727605993798306371900252997875213623046875]
      mask Display: e = 0.06;c1 = [120 150 230]/255;c2 = ([120 150 230]+0)/383;c3 = ([120 150 230]+128)/383;patch([0 1 1 0],[0 0 1 1],c1);patch([0 1 1 1-e 1-e 0+e],[0 0 1 1-e 0+e 0+e],c2);patch([0 0 1 1-e 0+e 0+e],[0 1 1 1-e 1-e 0+e],c3);plot([0 1 1 0 0],[0 0 1 1 0]);disp('Weights');
  "IW{1,1}(51,:)'" : Constant  Value=[0.9259942608069653413593869117903523147106170654296875;0.2834317478907593113035545684397220611572265625;-0.1896774579356290402198936817512731067836284637451171875;0.7903669928985408432708936743438243865966796875;0.72957881464813578720196574067813344299793243408203125;0.1866297045422728728691907917891512624919414520263671875;0.7587855195969968047364773156004957854747772216796875;1.21578580620694243208390616928227245807647705078125;-0.66228206929067223729390434527886100113391876220703125;-0.55062851824195024885710836315411143004894256591796875]
      mask Display: e = 0.06;c1 = [120 150 230]/255;c2 = ([120 150 230]+0)/383;c3 = ([120 150 230]+128)/383;patch([0 1 1 0],[0 0 1 1],c1);patch([0 1 1 1-e 1-e 0+e],[0 0 1 1-e 0+e 0+e],c2);patch([0 0 1 1-e 0+e 0+e],[0 1 1 1-e 1-e 0+e],c3);plot([0 1 1 0 0],[0 0 1 1 0]);disp('Weights');
  "IW{1,1}(52,:)'" : Constant  Value=[0.02002567052558699989273094388408935628831386566162109375;-0.210570773951820611191720900023938156664371490478515625;0.916153958310780947016382924630306661128997802734375;-0.9238043577369581260683162327040918171405792236328125;-0.026580037814816319385879950232265400700271129608154296875;-0.6301971954360607863776522208354435861110687255859375;-0.70717572182562082883094944918411783874034881591796875;0.8690171107075332912472731550224125385284423828125;0.8982399795902622496868161761085502803325653076171875;-0.72764750557503921069013586020446382462978363037109375]
      mask Display: e = 0.06;c1 = [120 150 230]/255;c2 = ([120 150 230]+0)/383;c3 = ([120 150 230]+128)/383;patch([0 1 1 0],[0 0 1 1],c1);patch([0 1 1 1-e 1-e 0+e],[0 0 1 1-e 0+e 0+e],c2);patch([0 0 1 1-e 0+e 0+e],[0 1 1 1-e 1-e 0+e],c3);plot([0 1 1 0 0],[0 0 1 1 0]);disp('Weights');
  "IW{1,1}(53,:)'" : Constant  Value=[-0.408499163126739006646204188655246980488300323486328125;1.001581821598624078006878335145302116870880126953125;-0.697825051389537431845155879273079335689544677734375;0.79773499815271176061060032225213944911956787109375;0.21346120470742457886359488838934339582920074462890625;0.6068901333816947296639909836812876164913177490234375;0.335070085875675383046967681366368196904659271240234375;-0.86574152681859029012656492341193370521068572998046875;-0.7689981105520591331270452428725548088550567626953125;-0.78656605784135091852249388466589152812957763671875]
      mask Display: e = 0.06;c1 = [120 150 230]/255;c2 = ([120 150 230]+0)/383;c3 = ([120 150 230]+128)/383;patch([0 1 1 0],[0 0 1 1],c1);patch([0 1 1 1-e 1-e 0+e],[0 0 1 1-e 0+e 0+e],c2);patch([0 0 1 1-e 0+e 0+e],[0 1 1 1-e 1-e 0+e],c3);plot([0 1 1 0 0],[0 0 1 1 0]);disp('Weights');
  "IW{1,1}(54,:)'" : Constant  Value=[-0.5597643817805109112129002824076451361179351806640625;1.2922610811795465224349754862487316131591796875;0.6148014658980993640824408430489711463451385498046875;-0.235131735683876963438621032764785923063755035400390625;0.6842293848715221837863964537973515689373016357421875;0.0842846991652959065532968452316708862781524658203125;-0.25966843985963283802931300670024938881397247314453125;0.63499870425546323104981638607569038867950439453125;0.67351327080654643797430480844923295080661773681640625;0.677975764070798181393229242530651390552520751953125]
      mask Display: e = 0.06;c1 = [120 150 230]/255;c2 = ([120 150 230]+0)/383;c3 = ([120 150 230]+128)/383;patch([0 1 1 0],[0 0 1 1],c1);patch([0 1 1 1-e 1-e 0+e],[0 0 1 1-e 0+e 0+e],c2);patch([0 0 1 1-e 0+e 0+e],[0 1 1 1-e 1-e 0+e],c3);plot([0 1 1 0 0],[0 0 1 1 0]);disp('Weights');
  "IW{1,1}(55,:)'" : Constant  Value=[-1.2639508142783946187392984938924200832843780517578125;0.36488131519973976413240279725869186222553253173828125;1.078849683991631280832734773866832256317138671875;0.30792969269853365243960752195562236011028289794921875;-0.315554412505322290360965098443557508289813995361328125;-0.0343026098416485403230780093508656136691570281982421875;0.105970207045530562250945649793720804154872894287109375;-0.1807066880430427124881731515415594913065433502197265625;-1.1977707022349000087757531218812800943851470947265625;-0.7838046300657024456626231767586432397365570068359375]
      mask Display: e = 0.06;c1 = [120 150 230]/255;c2 = ([120 150 230]+0)/383;c3 = ([120 150 230]+128)/383;patch([0 1 1 0],[0 0 1 1],c1);patch([0 1 1 1-e 1-e 0+e],[0 0 1 1-e 0+e 0+e],c2);patch([0 0 1 1-e 0+e 0+e],[0 1 1 1-e 1-e 0+e],c3);plot([0 1 1 0 0],[0 0 1 1 0]);disp('Weights');
  "IW{1,1}(56,:)'" : Constant  Value=[-0.091586787926671020532154443571926094591617584228515625;0.67707923818854054420768306954414583742618560791015625;-0.048050030168706424349434058740371256135404109954833984375;1.0154096269495074267297241021879017353057861328125;1.280405372086997228819882366224192082881927490234375;0.4756441844257228712677942894515581429004669189453125;0.02237284851160740994924225333306821994483470916748046875;0.3949019178514630024068310376605950295925140380859375;0.9302004608996712331503431414603255689144134521484375;-0.880200100827568387984456421690993010997772216796875]
      mask Display: e = 0.06;c1 = [120 150 230]/255;c2 = ([120 150 230]+0)/383;c3 = ([120 150 230]+128)/383;patch([0 1 1 0],[0 0 1 1],c1);patch([0 1 1 1-e 1-e 0+e],[0 0 1 1-e 0+e 0+e],c2);patch([0 0 1 1-e 0+e 0+e],[0 1 1 1-e 1-e 0+e],c3);plot([0 1 1 0 0],[0 0 1 1 0]);disp('Weights');
  "IW{1,1}(57,:)'" : Constant  Value=[0.4782932781060225124747375957667827606201171875;0.254402646522531250550258619114174507558345794677734375;0.60745032162029932720770375453867018222808837890625;1.073638874091563888413247696007601916790008544921875;0.3851798718466457049913742594071663916110992431640625;0.9052726227355216703784890341921709477901458740234375;0.8293298663679553595073912219959311187267303466796875;-0.83908778187295229855635625426657497882843017578125;0.44387714072731443426533814999856986105442047119140625;0.515093438395408664831620626500807702541351318359375]
      mask Display: e = 0.06;c1 = [120 150 230]/255;c2 = ([120 150 230]+0)/383;c3 = ([120 150 230]+128)/383;patch([0 1 1 0],[0 0 1 1],c1);patch([0 1 1 1-e 1-e 0+e],[0 0 1 1-e 0+e 0+e],c2);patch([0 0 1 1-e 0+e 0+e],[0 1 1 1-e 1-e 0+e],c3);plot([0 1 1 0 0],[0 0 1 1 0]);disp('Weights');
  "IW{1,1}(58,:)'" : Constant  Value=[-1.059069679671221120287327721598558127880096435546875;-0.26252777133790206054442251115688122808933258056640625;0.449913721433966184992669923303765244781970977783203125;0.667173504053206745112447606516070663928985595703125;-0.766345507458793928634577241609804332256317138671875;0.74240283931141359818894898126018233597278594970703125;-1.058869168911627411944209598004817962646484375;-0.419862823221478553836760738704469986259937286376953125;-0.6939041477028322635334234291804023087024688720703125;-0.77337158079841950009125639553531073033809661865234375]
      mask Display: e = 0.06;c1 = [120 150 230]/255;c2 = ([120 150 230]+0)/383;c3 = ([120 150 230]+128)/383;patch([0 1 1 0],[0 0 1 1],c1);patch([0 1 1 1-e 1-e 0+e],[0 0 1 1-e 0+e 0+e],c2);patch([0 0 1 1-e 0+e 0+e],[0 1 1 1-e 1-e 0+e],c3);plot([0 1 1 0 0],[0 0 1 1 0]);disp('Weights');
  "IW{1,1}(59,:)'" : Constant  Value=[-0.651976950718070380474955527461133897304534912109375;0.9541726237996270842955937041551806032657623291015625;-0.6230203651029946332329245706205256283283233642578125;0.79703637277315364517704665558994747698307037353515625;0.343456871388214401985550239260192029178142547607421875;-0.8830029755329265039875963339000009000301361083984375;0.023094574423245417538197443718672730028629302978515625;-0.77393362574773127970928499053115956485271453857421875;0.5295498392763546835482202368439175188541412353515625;-0.87070875851380546972535512395552359521389007568359375]
      mask Display: e = 0.06;c1 = [120 150 230]/255;c2 = ([120 150 230]+0)/383;c3 = ([120 150 230]+128)/383;patch([0 1 1 0],[0 0 1 1],c1);patch([0 1 1 1-e 1-e 0+e],[0 0 1 1-e 0+e 0+e],c2);patch([0 0 1 1-e 0+e 0+e],[0 1 1 1-e 1-e 0+e],c3);plot([0 1 1 0 0],[0 0 1 1 0]);disp('Weights');
  "IW{1,1}(6,:)'" : Constant  Value=[-0.358338106226035513213190597525681369006633758544921875;-0.62887308907696104487428101492696441709995269775390625;-0.7263535051120662000556649218196980655193328857421875;0.81047815383696064639451606126385740935802459716796875;-0.65980237470839508961972796896588988602161407470703125;0.85842590182956601818631270361947827041149139404296875;0.340937112989122825812415840118774212896823883056640625;-1.0066521690828247326265909578069113194942474365234375;-0.79426115224283166948993084588437341153621673583984375;0.12436518431718744659431052923537208698689937591552734375]
      mask Display: e = 0.06;c1 = [120 150 230]/255;c2 = ([120 150 230]+0)/383;c3 = ([120 150 230]+128)/383;patch([0 1 1 0],[0 0 1 1],c1);patch([0 1 1 1-e 1-e 0+e],[0 0 1 1-e 0+e 0+e],c2);patch([0 0 1 1-e 0+e 0+e],[0 1 1 1-e 1-e 0+e],c3);plot([0 1 1 0 0],[0 0 1 1 0]);disp('Weights');
  "IW{1,1}(60,:)'" : Constant  Value=[1.0419211638783298923272013780660927295684814453125;0.01241633102607135781536573659877831232734024524688720703125;-0.999564149777570687405159333138726651668548583984375;0.6146978196383710013606105349026620388031005859375;1.0840737945441694112247432713047601282596588134765625;-0.9285164983940139560303350663161836564540863037109375;-0.0488649367132618361875273649275186471641063690185546875;-0.10557057229641397810837588622234761714935302734375;0.224208746001478720355493123861378990113735198974609375;-0.7441530249885615067029220881522633135318756103515625]
      mask Display: e = 0.06;c1 = [120 150 230]/255;c2 = ([120 150 230]+0)/383;c3 = ([120 150 230]+128)/383;patch([0 1 1 0],[0 0 1 1],c1);patch([0 1 1 1-e 1-e 0+e],[0 0 1 1-e 0+e 0+e],c2);patch([0 0 1 1-e 0+e 0+e],[0 1 1 1-e 1-e 0+e],c3);plot([0 1 1 0 0],[0 0 1 1 0]);disp('Weights');
  "IW{1,1}(61,:)'" : Constant  Value=[-1.36232620688122540997255782713182270526885986328125;0.98414955750769317344150977078243158757686614990234375;0.257092122139868928254458069204702042043209075927734375;-0.58187529626702794161019482999108731746673583984375;-0.4823360093755668653869861373095773160457611083984375;0.037664407871627114676726932884776033461093902587890625;-0.465825973080071731313722693812451325356960296630859375;0.58583310891078299587064748266129754483699798583984375;-0.07949808409345686388558505086621153168380260467529296875;0.94669178922415475607721191408927552402019500732421875]
      mask Display: e = 0.06;c1 = [120 150 230]/255;c2 = ([120 150 230]+0)/383;c3 = ([120 150 230]+128)/383;patch([0 1 1 0],[0 0 1 1],c1);patch([0 1 1 1-e 1-e 0+e],[0 0 1 1-e 0+e 0+e],c2);patch([0 0 1 1-e 0+e 0+e],[0 1 1 1-e 1-e 0+e],c3);plot([0 1 1 0 0],[0 0 1 1 0]);disp('Weights');
  "IW{1,1}(62,:)'" : Constant  Value=[-0.78528950077653114636433429041062481701374053955078125;-0.6254668709558381944901839233352802693843841552734375;0.96779939070130127642954676048248074948787689208984375;0.08874771663928983367330971532283001579344272613525390625;0.224989917402083905439980071605532430112361907958984375;0.496312795904943815372689641662873327732086181640625;0.563910104544832702089252052246592938899993896484375;0.8049792488463409778631785229663364589214324951171875;-0.7573746698149605993677369042416103184223175048828125;-0.91856189193760340305772160718333907425403594970703125]
      mask Display: e = 0.06;c1 = [120 150 230]/255;c2 = ([120 150 230]+0)/383;c3 = ([120 150 230]+128)/383;patch([0 1 1 0],[0 0 1 1],c1);patch([0 1 1 1-e 1-e 0+e],[0 0 1 1-e 0+e 0+e],c2);patch([0 0 1 1-e 0+e 0+e],[0 1 1 1-e 1-e 0+e],c3);plot([0 1 1 0 0],[0 0 1 1 0]);disp('Weights');
  "IW{1,1}(63,:)'" : Constant  Value=[0.786316276607621045258156300405971705913543701171875;0.79545825613742671134076545058633200824260711669921875;0.369355258487485738072564345202408730983734130859375;-0.964140766585051434134356895810924470424652099609375;0.80125399297140942334038982153288088738918304443359375;0.80314455348714408611243698032922111451625823974609375;-0.57858090995740230066957110466319136321544647216796875;-0.60366181263723195371539986808784306049346923828125;0.75851920767219238594947228193632327020168304443359375;0.458335171065112623178805506540811620652675628662109375]
      mask Display: e = 0.06;c1 = [120 150 230]/255;c2 = ([120 150 230]+0)/383;c3 = ([120 150 230]+128)/383;patch([0 1 1 0],[0 0 1 1],c1);patch([0 1 1 1-e 1-e 0+e],[0 0 1 1-e 0+e 0+e],c2);patch([0 0 1 1-e 0+e 0+e],[0 1 1 1-e 1-e 0+e],c3);plot([0 1 1 0 0],[0 0 1 1 0]);disp('Weights');
  "IW{1,1}(64,:)'" : Constant  Value=[-0.270406431548540104881084289445425383746623992919921875;1.160328119424433257478312953026033937931060791015625;0.41476213234578274136055142662371508777141571044921875;-0.995490848833870956013925024308264255523681640625;-0.01156545385676677369091169822468145866878330707550048828125;-1.0644174728225166415285229959408752620220184326171875;-0.394804764473468738916750453427084721624851226806640625;0.196163989704971564176361198406084440648555755615234375;-0.453171520765595137181236395917949266731739044189453125;-0.85144751603115242932773298889514990150928497314453125]
      mask Display: e = 0.06;c1 = [120 150 230]/255;c2 = ([120 150 230]+0)/383;c3 = ([120 150 230]+128)/383;patch([0 1 1 0],[0 0 1 1],c1);patch([0 1 1 1-e 1-e 0+e],[0 0 1 1-e 0+e 0+e],c2);patch([0 0 1 1-e 0+e 0+e],[0 1 1 1-e 1-e 0+e],c3);plot([0 1 1 0 0],[0 0 1 1 0]);disp('Weights');
  "IW{1,1}(65,:)'" : Constant  Value=[1.163006902052404978320510053890757262706756591796875;0.576397616734676265792813865118660032749176025390625;-0.1166018102222483865393343194227782078087329864501953125;-1.1591611771860554913615715122432447969913482666015625;0.58878185106495439793405921591329388320446014404296875;-0.384119831188158122881048939234460704028606414794921875;-0.54715160606758794781256938222213648259639739990234375;1.1084013902385307925868573875050060451030731201171875;0.03239991618314345955820243716516415588557720184326171875;-0.1290575331341615450408966125905863009393215179443359375]
      mask Display: e = 0.06;c1 = [120 150 230]/255;c2 = ([120 150 230]+0)/383;c3 = ([120 150 230]+128)/383;patch([0 1 1 0],[0 0 1 1],c1);patch([0 1 1 1-e 1-e 0+e],[0 0 1 1-e 0+e 0+e],c2);patch([0 0 1 1-e 0+e 0+e],[0 1 1 1-e 1-e 0+e],c3);plot([0 1 1 0 0],[0 0 1 1 0]);disp('Weights');
  "IW{1,1}(66,:)'" : Constant  Value=[-0.293147766109261020961440635801409371197223663330078125;0.8519170627905057191497917301603592932224273681640625;1.0780899459296648945638708028127439320087432861328125;-0.2291434532938055046447090035144356079399585723876953125;-0.723877741435821508986236949567683041095733642578125;-0.91089592778029315756072037402191199362277984619140625;0.08078532726024378884943644152372144162654876708984375;0.469691348270626918282033557261456735432147979736328125;0.784604489771459245872620158479548990726470947265625;0.71526753691329625350903143043979071080684661865234375]
      mask Display: e = 0.06;c1 = [120 150 230]/255;c2 = ([120 150 230]+0)/383;c3 = ([120 150 230]+128)/383;patch([0 1 1 0],[0 0 1 1],c1);patch([0 1 1 1-e 1-e 0+e],[0 0 1 1-e 0+e 0+e],c2);patch([0 0 1 1-e 0+e 0+e],[0 1 1 1-e 1-e 0+e],c3);plot([0 1 1 0 0],[0 0 1 1 0]);disp('Weights');
  "IW{1,1}(67,:)'" : Constant  Value=[1.0624460469624528169418908873922191560268402099609375;-0.7551030070212221279035702536930330097675323486328125;-0.0110930898180549297737940150909707881510257720947265625;-0.19448594236993610451236236258409917354583740234375;-0.70915741516854280401815913137397728860378265380859375;0.366754741228828062826750056046876125037670135498046875;0.942761827410462327492268741480074822902679443359375;0.8593984772859959431201559709734283387660980224609375;0.81178735778599564465451976502663455903530120849609375;-0.87252681560695022344731341945589520037174224853515625]
      mask Display: e = 0.06;c1 = [120 150 230]/255;c2 = ([120 150 230]+0)/383;c3 = ([120 150 230]+128)/383;patch([0 1 1 0],[0 0 1 1],c1);patch([0 1 1 1-e 1-e 0+e],[0 0 1 1-e 0+e 0+e],c2);patch([0 0 1 1-e 0+e 0+e],[0 1 1 1-e 1-e 0+e],c3);plot([0 1 1 0 0],[0 0 1 1 0]);disp('Weights');
  "IW{1,1}(68,:)'" : Constant  Value=[0.88380536529908948484290931446594186127185821533203125;0.0881799524145983060208209280972369015216827392578125;0.0471792699202187304496902697792393155395984649658203125;-0.1468570015303254649996489433760871179401874542236328125;0.73241035771120788222532382860663346946239471435546875;-1.412205356097323782904595645959489047527313232421875;-0.54444514761401119340433751858654431998729705810546875;0.6837134821129300377151594148017466068267822265625;-0.56806333308878576016098804757348261773586273193359375;0.782565530792702634954594032024033367633819580078125]
      mask Display: e = 0.06;c1 = [120 150 230]/255;c2 = ([120 150 230]+0)/383;c3 = ([120 150 230]+128)/383;patch([0 1 1 0],[0 0 1 1],c1);patch([0 1 1 1-e 1-e 0+e],[0 0 1 1-e 0+e 0+e],c2);patch([0 0 1 1-e 0+e 0+e],[0 1 1 1-e 1-e 0+e],c3);plot([0 1 1 0 0],[0 0 1 1 0]);disp('Weights');
  "IW{1,1}(69,:)'" : Constant  Value=[-0.5337571784352583836863459509913809597492218017578125;0.366932000711891692645849616383202373981475830078125;0.27584666055029949394139521245961077511310577392578125;-1.11809985503576836407546579721383750438690185546875;-0.57789075622623709005409864403191022574901580810546875;-0.86413426384765756882444520670105703175067901611328125;-0.6766885741782078245165621410706080496311187744140625;-0.06656805809616099522951770950385252945125102996826171875;-0.87698238604058642575722615220001898705959320068359375;-0.84212634448051792990241892766789533197879791259765625]
      mask Display: e = 0.06;c1 = [120 150 230]/255;c2 = ([120 150 230]+0)/383;c3 = ([120 150 230]+128)/383;patch([0 1 1 0],[0 0 1 1],c1);patch([0 1 1 1-e 1-e 0+e],[0 0 1 1-e 0+e 0+e],c2);patch([0 0 1 1-e 0+e 0+e],[0 1 1 1-e 1-e 0+e],c3);plot([0 1 1 0 0],[0 0 1 1 0]);disp('Weights');
  "IW{1,1}(7,:)'" : Constant  Value=[0.23582185959203816327800495855626650154590606689453125;-0.12825009716719326657852207063115201890468597412109375;-0.24645434161327661737317384904599748551845550537109375;-0.5626490043075176306075491083902306854724884033203125;-1.2933279169817648579510205308906733989715576171875;0.59789483021397737960711538107716478407382965087890625;-1.0901093982971927776048914893181063234806060791015625;0.54585860231715865875656845673802308738231658935546875;0.950354705523938303457498477655462920665740966796875;0.86014287558777080544558657493325881659984588623046875]
      mask Display: e = 0.06;c1 = [120 150 230]/255;c2 = ([120 150 230]+0)/383;c3 = ([120 150 230]+128)/383;patch([0 1 1 0],[0 0 1 1],c1);patch([0 1 1 1-e 1-e 0+e],[0 0 1 1-e 0+e 0+e],c2);patch([0 0 1 1-e 0+e 0+e],[0 1 1 1-e 1-e 0+e],c3);plot([0 1 1 0 0],[0 0 1 1 0]);disp('Weights');
  "IW{1,1}(70,:)'" : Constant  Value=[-0.420718462404398862997112473749439232051372528076171875;-0.97368581714669921733928958929027430713176727294921875;0.4179798543378385744517800048924982547760009765625;0.092068767351608793436668065623962320387363433837890625;0.61762547982337867580326928873546421527862548828125;-0.8439735181314216294623520298046059906482696533203125;-0.1501507923868820870705320658089476637542247772216796875;-0.72311513680753070065776455521699972450733184814453125;-0.92909385148707956947333741481998004019260406494140625;-0.59421770688347042010946097434498369693756103515625]
      mask Display: e = 0.06;c1 = [120 150 230]/255;c2 = ([120 150 230]+0)/383;c3 = ([120 150 230]+128)/383;patch([0 1 1 0],[0 0 1 1],c1);patch([0 1 1 1-e 1-e 0+e],[0 0 1 1-e 0+e 0+e],c2);patch([0 0 1 1-e 0+e 0+e],[0 1 1 1-e 1-e 0+e],c3);plot([0 1 1 0 0],[0 0 1 1 0]);disp('Weights');
  "IW{1,1}(71,:)'" : Constant  Value=[-0.042545331350925356950209987871858174912631511688232421875;0.11741457175703706727887265515164472162723541259765625;-0.69538726926277727447001097971224226057529449462890625;-0.255134987463223439352333343776990659534931182861328125;-0.216666459981731673867244580833357758820056915283203125;-0.98796252115794247483648859997629188001155853271484375;-1.0484171472878822672925025472068227827548980712890625;0.94809287165744304815007126308046281337738037109375;-0.8312002469229351486745827060076408088207244873046875;1.006182705877052274701100031961686909198760986328125]
      mask Display: e = 0.06;c1 = [120 150 230]/255;c2 = ([120 150 230]+0)/383;c3 = ([120 150 230]+128)/383;patch([0 1 1 0],[0 0 1 1],c1);patch([0 1 1 1-e 1-e 0+e],[0 0 1 1-e 0+e 0+e],c2);patch([0 0 1 1-e 0+e 0+e],[0 1 1 1-e 1-e 0+e],c3);plot([0 1 1 0 0],[0 0 1 1 0]);disp('Weights');
  "IW{1,1}(72,:)'" : Constant  Value=[-0.7780460130054003276001139965956099331378936767578125;0.1892914475513987060395493244868703186511993408203125;0.329723677999647579728303981028147973120212554931640625;-0.3475498163809682683478285980527289211750030517578125;-0.69568895337473668494254752658889628946781158447265625;1.0653235191647374424661620651022531092166900634765625;0.332026813462277858857163437278359197080135345458984375;-0.5283746137775562345950675080530345439910888671875;1.086395743126612689621879326296038925647735595703125;0.94096689557850765606161758114467374980449676513671875]
      mask Display: e = 0.06;c1 = [120 150 230]/255;c2 = ([120 150 230]+0)/383;c3 = ([120 150 230]+128)/383;patch([0 1 1 0],[0 0 1 1],c1);patch([0 1 1 1-e 1-e 0+e],[0 0 1 1-e 0+e 0+e],c2);patch([0 0 1 1-e 0+e 0+e],[0 1 1 1-e 1-e 0+e],c3);plot([0 1 1 0 0],[0 0 1 1 0]);disp('Weights');
  "IW{1,1}(73,:)'" : Constant  Value=[0.98578013307484047000883720102137885987758636474609375;-1.03668845795895681050069470074959099292755126953125;-0.416663073849689313821187397479661740362644195556640625;0.8819376144881461154767521293251775205135345458984375;-0.67770433822329378958926326959044672548770904541015625;0.01482599579637229776640783285301949945278465747833251953125;0.302670983494109757661050252863788045942783355712890625;0.325497259307157893459816477843560278415679931640625;1.0574248262699106337692001034156419336795806884765625;0.8412204169647434781609263154678046703338623046875]
      mask Display: e = 0.06;c1 = [120 150 230]/255;c2 = ([120 150 230]+0)/383;c3 = ([120 150 230]+128)/383;patch([0 1 1 0],[0 0 1 1],c1);patch([0 1 1 1-e 1-e 0+e],[0 0 1 1-e 0+e 0+e],c2);patch([0 0 1 1-e 0+e 0+e],[0 1 1 1-e 1-e 0+e],c3);plot([0 1 1 0 0],[0 0 1 1 0]);disp('Weights');
  "IW{1,1}(74,:)'" : Constant  Value=[1.0109822412469513519539532353519462049007415771484375;-0.85795572138731979183745579575770534574985504150390625;0.64598381289388784320948388995020650327205657958984375;-0.13281236949030217342482274034409783780574798583984375;-0.51629731789295529864602940506301820278167724609375;-0.96955795008787115651927024373435415327548980712890625;-0.881928194150545241569716381491161882877349853515625;-0.3303051680192898853505312217748723924160003662109375;-0.3450132593593517871255471618496812880039215087890625;0.5702957718727892366672449497855268418788909912109375]
      mask Display: e = 0.06;c1 = [120 150 230]/255;c2 = ([120 150 230]+0)/383;c3 = ([120 150 230]+128)/383;patch([0 1 1 0],[0 0 1 1],c1);patch([0 1 1 1-e 1-e 0+e],[0 0 1 1-e 0+e 0+e],c2);patch([0 0 1 1-e 0+e 0+e],[0 1 1 1-e 1-e 0+e],c3);plot([0 1 1 0 0],[0 0 1 1 0]);disp('Weights');
  "IW{1,1}(75,:)'" : Constant  Value=[-1.05755595751302422513617784716188907623291015625;-0.8082419283354991268453204611432738602161407470703125;-0.292746138196071481463178542981040664017200469970703125;-0.87280165496597106322695935887168161571025848388671875;0.74524114908454208716648281551897525787353515625;0.74287002935675838788398550605052150785923004150390625;0.695910793947912775792019601794891059398651123046875;0.5862132279634841847126836000825278460979461669921875;0.504490293599527461765319458208978176116943359375;-0.1768113009116248079966027262344141490757465362548828125]
      mask Display: e = 0.06;c1 = [120 150 230]/255;c2 = ([120 150 230]+0)/383;c3 = ([120 150 230]+128)/383;patch([0 1 1 0],[0 0 1 1],c1);patch([0 1 1 1-e 1-e 0+e],[0 0 1 1-e 0+e 0+e],c2);patch([0 0 1 1-e 0+e 0+e],[0 1 1 1-e 1-e 0+e],c3);plot([0 1 1 0 0],[0 0 1 1 0]);disp('Weights');
  "IW{1,1}(76,:)'" : Constant  Value=[0.61019896492028269374685578441130928695201873779296875;0.740489934030562846345446814666502177715301513671875;0.081939707389603377851727827874128706753253936767578125;-0.88647318479788939082908427735674194991588592529296875;-0.7452659025752261801045506217633374035358428955078125;-0.58652885785380670657929158551269210875034332275390625;-0.015978363949191880244438124236694420687854290008544921875;-0.9740225273453397836220801764284260571002960205078125;-0.976958582638513650664435772341676056385040283203125;0.4370131592679136200985112736816518008708953857421875]
      mask Display: e = 0.06;c1 = [120 150 230]/255;c2 = ([120 150 230]+0)/383;c3 = ([120 150 230]+128)/383;patch([0 1 1 0],[0 0 1 1],c1);patch([0 1 1 1-e 1-e 0+e],[0 0 1 1-e 0+e 0+e],c2);patch([0 0 1 1-e 0+e 0+e],[0 1 1 1-e 1-e 0+e],c3);plot([0 1 1 0 0],[0 0 1 1 0]);disp('Weights');
  "IW{1,1}(77,:)'" : Constant  Value=[-0.559090537644634455460845856578089296817779541015625;0.08839443579741652901038406753286835737526416778564453125;0.14158763272424135237770315143279731273651123046875;0.9182980981039203793869774017366580665111541748046875;-0.94400429769697702386821447362308390438556671142578125;-1.005288764253680522386957818525843322277069091796875;-0.61826810136142384966007057300885207951068878173828125;1.0312628046617413613006419836892746388912200927734375;0.31842374678058382730938546956167556345462799072265625;0.412337990287018840707133904288639314472675323486328125]
      mask Display: e = 0.06;c1 = [120 150 230]/255;c2 = ([120 150 230]+0)/383;c3 = ([120 150 230]+128)/383;patch([0 1 1 0],[0 0 1 1],c1);patch([0 1 1 1-e 1-e 0+e],[0 0 1 1-e 0+e 0+e],c2);patch([0 0 1 1-e 0+e 0+e],[0 1 1 1-e 1-e 0+e],c3);plot([0 1 1 0 0],[0 0 1 1 0]);disp('Weights');
  "IW{1,1}(78,:)'" : Constant  Value=[0.4996910957834106437047694271313957870006561279296875;-0.82905154565432248592316000213031657040119171142578125;-0.56900587555671100492560299244360066950321197509765625;-0.321587039590590484383625380360172130167484283447265625;0.88412689519616216582420520353480242192745208740234375;0.9640577708151314428874911754974164068698883056640625;0.915961760985546380453570236568339169025421142578125;-0.221661940765695675281676813028752803802490234375;0.7514481944043012173750639703939668834209442138671875;-0.463014694920261760113788795933942310512065887451171875]
      mask Display: e = 0.06;c1 = [120 150 230]/255;c2 = ([120 150 230]+0)/383;c3 = ([120 150 230]+128)/383;patch([0 1 1 0],[0 0 1 1],c1);patch([0 1 1 1-e 1-e 0+e],[0 0 1 1-e 0+e 0+e],c2);patch([0 0 1 1-e 0+e 0+e],[0 1 1 1-e 1-e 0+e],c3);plot([0 1 1 0 0],[0 0 1 1 0]);disp('Weights');
  "IW{1,1}(79,:)'" : Constant  Value=[-0.174287652221410682695790228535770438611507415771484375;-1.006197513095864248811039942665956914424896240234375;-1.1361891256292342422540286861476488411426544189453125;0.99880992155110959185293495465884916484355926513671875;0.448178182092145827031259841533028520643711090087890625;0.392234919317140884320593841039226390421390533447265625;-0.60056920435631899746198314460343681275844573974609375;-0.65549287731696537218084586129407398402690887451171875;-0.37884253709052539971224859982612542808055877685546875;0.3410403531269599053388219545013271272182464599609375]
      mask Display: e = 0.06;c1 = [120 150 230]/255;c2 = ([120 150 230]+0)/383;c3 = ([120 150 230]+128)/383;patch([0 1 1 0],[0 0 1 1],c1);patch([0 1 1 1-e 1-e 0+e],[0 0 1 1-e 0+e 0+e],c2);patch([0 0 1 1-e 0+e 0+e],[0 1 1 1-e 1-e 0+e],c3);plot([0 1 1 0 0],[0 0 1 1 0]);disp('Weights');
  "IW{1,1}(8,:)'" : Constant  Value=[-0.75715661668662692651565748747088946402072906494140625;0.57222087234582108550284829107113182544708251953125;0.9110287483878283243399209823110140860080718994140625;0.45501542110246473438195380367687903344631195068359375;0.45310650580574785006859883651486597955226898193359375;-0.71341866578888291083870853981352411210536956787109375;0.21969355042121418986056369249126873910427093505859375;0.43896900974833241715344911426655016839504241943359375;-1.36761128842876278355333852232433855533599853515625;-0.08903709242504458110101239753930713050067424774169921875]
      mask Display: e = 0.06;c1 = [120 150 230]/255;c2 = ([120 150 230]+0)/383;c3 = ([120 150 230]+128)/383;patch([0 1 1 0],[0 0 1 1],c1);patch([0 1 1 1-e 1-e 0+e],[0 0 1 1-e 0+e 0+e],c2);patch([0 0 1 1-e 0+e 0+e],[0 1 1 1-e 1-e 0+e],c3);plot([0 1 1 0 0],[0 0 1 1 0]);disp('Weights');
  "IW{1,1}(80,:)'" : Constant  Value=[0.93415019403994870028640207237913273274898529052734375;0.83393923005527437197770268539898097515106201171875;0.31657674069495389534978357914951629936695098876953125;-1.1727727685552764569365535862743854522705078125;0.74068925435657206879369596208562143146991729736328125;-0.324281218774995938503025172394700348377227783203125;-0.34950992335420938417200886760838329792022705078125;0.432253956796601224166209931354387663304805755615234375;0.8799110172299562382391968640149571001529693603515625;0.0268827998771871169714220428659245953895151615142822265625]
      mask Display: e = 0.06;c1 = [120 150 230]/255;c2 = ([120 150 230]+0)/383;c3 = ([120 150 230]+128)/383;patch([0 1 1 0],[0 0 1 1],c1);patch([0 1 1 1-e 1-e 0+e],[0 0 1 1-e 0+e 0+e],c2);patch([0 0 1 1-e 0+e 0+e],[0 1 1 1-e 1-e 0+e],c3);plot([0 1 1 0 0],[0 0 1 1 0]);disp('Weights');
  "IW{1,1}(81,:)'" : Constant  Value=[-0.2731397225651706062166113042621873319149017333984375;0.85972472528934773539077696113963611423969268798828125;1.0058686746294893676889614653191529214382171630859375;-0.69351826878154942956911099827266298234462738037109375;0.263158726804439024871129504390410147607326507568359375;0.0315794066412405094457227505699847824871540069580078125;-0.834199394123601223327568732202053070068359375;-0.61433065473817516366494828616851009428501129150390625;0.62385437771374008253388865341548807919025421142578125;0.948607897626992713213667229865677654743194580078125]
      mask Display: e = 0.06;c1 = [120 150 230]/255;c2 = ([120 150 230]+0)/383;c3 = ([120 150 230]+128)/383;patch([0 1 1 0],[0 0 1 1],c1);patch([0 1 1 1-e 1-e 0+e],[0 0 1 1-e 0+e 0+e],c2);patch([0 0 1 1-e 0+e 0+e],[0 1 1 1-e 1-e 0+e],c3);plot([0 1 1 0 0],[0 0 1 1 0]);disp('Weights');
  "IW{1,1}(82,:)'" : Constant  Value=[1.2961048448220642281825121244764886796474456787109375;-0.6935852974641687485046759320539422333240509033203125;-0.92125842493590892612331799682579003274440765380859375;0.8630251704283191660493912422680296003818511962890625;-0.80705039628131469697791544604115188121795654296875;0.95813657998923584813155684969387948513031005859375;-0.387262167368896237373832036610110662877559661865234375;0.57125527671745823798943320070975460112094879150390625;-0.6157459038015196117754612714634276926517486572265625;0.0223709614910606834070616599774439237080514430999755859375]
      mask Display: e = 0.06;c1 = [120 150 230]/255;c2 = ([120 150 230]+0)/383;c3 = ([120 150 230]+128)/383;patch([0 1 1 0],[0 0 1 1],c1);patch([0 1 1 1-e 1-e 0+e],[0 0 1 1-e 0+e 0+e],c2);patch([0 0 1 1-e 0+e 0+e],[0 1 1 1-e 1-e 0+e],c3);plot([0 1 1 0 0],[0 0 1 1 0]);disp('Weights');
  "IW{1,1}(83,:)'" : Constant  Value=[-1.1751222607008908749293141227099113166332244873046875;0.1500297175647094249928414910755236633121967315673828125;0.274924117071083717878110519450274296104907989501953125;-0.85413103073990159774808716974803246557712554931640625;0.289345982762631848128620504212449304759502410888671875;-0.32704914736164647504068625494255684316158294677734375;-0.722828932066496232522467835224233567714691162109375;-0.423506969662987564628764403096283785998821258544921875;1.4234613372634168371178020606748759746551513671875;0.054627128694978488443467767865513451397418975830078125]
      mask Display: e = 0.06;c1 = [120 150 230]/255;c2 = ([120 150 230]+0)/383;c3 = ([120 150 230]+128)/383;patch([0 1 1 0],[0 0 1 1],c1);patch([0 1 1 1-e 1-e 0+e],[0 0 1 1-e 0+e 0+e],c2);patch([0 0 1 1-e 0+e 0+e],[0 1 1 1-e 1-e 0+e],c3);plot([0 1 1 0 0],[0 0 1 1 0]);disp('Weights');
  "IW{1,1}(84,:)'" : Constant  Value=[0.1607672715976770916324056770463357679545879364013671875;0.06979179056947959480794452247209846973419189453125;-0.83878374152797352536481412244029343128204345703125;-0.429619357578148342025059491788852028548717498779296875;1.0315884801148385019331499279360286891460418701171875;-0.16320249177149237507222778731375001370906829833984375;1.0266733347197660730643065107869915664196014404296875;-1.3060856491849011096206822912790812551975250244140625;0.1996025914800399758686211271196953020989894866943359375;0.10161514073787390743941472237565903924405574798583984375]
      mask Display: e = 0.06;c1 = [120 150 230]/255;c2 = ([120 150 230]+0)/383;c3 = ([120 150 230]+128)/383;patch([0 1 1 0],[0 0 1 1],c1);patch([0 1 1 1-e 1-e 0+e],[0 0 1 1-e 0+e 0+e],c2);patch([0 0 1 1-e 0+e 0+e],[0 1 1 1-e 1-e 0+e],c3);plot([0 1 1 0 0],[0 0 1 1 0]);disp('Weights');
  "IW{1,1}(85,:)'" : Constant  Value=[0.57020813290714211785115139718982391059398651123046875;1.008004058373262790127000698703341186046600341796875;0.608725400570859331850215312442742288112640380859375;0.30707972743389955194714957542601041495800018310546875;1.122618033053293107315084853325970470905303955078125;-0.47241649763107085302493715062155388295650482177734375;0.36066385502693709685928524777409620583057403564453125;0.7328384760560096022885545608005486428737640380859375;0.1787635059458099473506109688969445414841175079345703125;0.91516015653622873049499730768729932606220245361328125]
      mask Display: e = 0.06;c1 = [120 150 230]/255;c2 = ([120 150 230]+0)/383;c3 = ([120 150 230]+128)/383;patch([0 1 1 0],[0 0 1 1],c1);patch([0 1 1 1-e 1-e 0+e],[0 0 1 1-e 0+e 0+e],c2);patch([0 0 1 1-e 0+e 0+e],[0 1 1 1-e 1-e 0+e],c3);plot([0 1 1 0 0],[0 0 1 1 0]);disp('Weights');
  "IW{1,1}(86,:)'" : Constant  Value=[0.472654795850441844518030620747595094144344329833984375;-0.50776505347523925859576365837710909545421600341796875;0.7682297927957846273017139537842012941837310791015625;0.32941376472370664796329720047651790082454681396484375;0.64199002888989975534883569707744754850864410400390625;-1.00816374902594585449833175516687333583831787109375;-0.12037833035227775424491625244627357460558414459228515625;0.80556711500824895733074981762911193072795867919921875;-0.9829643134782148905514986836351454257965087890625;-0.686119333988397528401037561707198619842529296875]
      mask Display: e = 0.06;c1 = [120 150 230]/255;c2 = ([120 150 230]+0)/383;c3 = ([120 150 230]+128)/383;patch([0 1 1 0],[0 0 1 1],c1);patch([0 1 1 1-e 1-e 0+e],[0 0 1 1-e 0+e 0+e],c2);patch([0 0 1 1-e 0+e 0+e],[0 1 1 1-e 1-e 0+e],c3);plot([0 1 1 0 0],[0 0 1 1 0]);disp('Weights');
  "IW{1,1}(87,:)'" : Constant  Value=[-0.08690133063218559439366828200945747084915637969970703125;-0.84215994250171000157223488713498227298259735107421875;-0.043030184374000406133387031104575726203620433807373046875;0.72295678613017588798328461052733473479747772216796875;1.249763528259489220317846047692000865936279296875;0.46545418678936101297693994638393633067607879638671875;0.75851317328839840126164517641882412135601043701171875;0.849884700380383772966297328821383416652679443359375;-0.4639853986197317592399258501245640218257904052734375;0.05691949307353734444081538867976632900536060333251953125]
      mask Display: e = 0.06;c1 = [120 150 230]/255;c2 = ([120 150 230]+0)/383;c3 = ([120 150 230]+128)/383;patch([0 1 1 0],[0 0 1 1],c1);patch([0 1 1 1-e 1-e 0+e],[0 0 1 1-e 0+e 0+e],c2);patch([0 0 1 1-e 0+e 0+e],[0 1 1 1-e 1-e 0+e],c3);plot([0 1 1 0 0],[0 0 1 1 0]);disp('Weights');
  "IW{1,1}(88,:)'" : Constant  Value=[-0.558030025979658450552278736722655594348907470703125;-0.2877798741548023286895841010846197605133056640625;-0.698269222460341953961915351101197302341461181640625;-0.466400625773120136585703221498988568782806396484375;0.971534947990547070872935364604927599430084228515625;-0.0516907093470966305659430872765369713306427001953125;-0.34455215363270952355634335617651231586933135986328125;0.82950280562583678101162831808323971927165985107421875;1.1219110410438404290545122421463020145893096923828125;-0.90176054056776500100767179901595227420330047607421875]
      mask Display: e = 0.06;c1 = [120 150 230]/255;c2 = ([120 150 230]+0)/383;c3 = ([120 150 230]+128)/383;patch([0 1 1 0],[0 0 1 1],c1);patch([0 1 1 1-e 1-e 0+e],[0 0 1 1-e 0+e 0+e],c2);patch([0 0 1 1-e 0+e 0+e],[0 1 1 1-e 1-e 0+e],c3);plot([0 1 1 0 0],[0 0 1 1 0]);disp('Weights');
  "IW{1,1}(89,:)'" : Constant  Value=[0.79567551046389528579538819030858576297760009765625;0.01449725514493583992947645100457521039061248302459716796875;0.9310640672732670708455771091394126415252685546875;0.7597145208815228034637812015716917812824249267578125;-0.72315621675991081929169013164937496185302734375;0.395678902897997175625022236999939195811748504638671875;0.77022057836290602761408763399231247603893280029296875;-0.6730404049676319555572945318999700248241424560546875;-0.33277488088002693533695719452225603163242340087890625;0.98251613397519321768669442462851293385028839111328125]
      mask Display: e = 0.06;c1 = [120 150 230]/255;c2 = ([120 150 230]+0)/383;c3 = ([120 150 230]+128)/383;patch([0 1 1 0],[0 0 1 1],c1);patch([0 1 1 1-e 1-e 0+e],[0 0 1 1-e 0+e 0+e],c2);patch([0 0 1 1-e 0+e 0+e],[0 1 1 1-e 1-e 0+e],c3);plot([0 1 1 0 0],[0 0 1 1 0]);disp('Weights');
  "IW{1,1}(9,:)'" : Constant  Value=[0.64836613598423731286146676211501471698284149169921875;-0.84486682685632763512018073015497066080570220947265625;0.4507408080613914957979204700677655637264251708984375;0.056906996154878243532326820286471047438681125640869140625;0.2025009578838637691600155221749446354806423187255859375;-0.373401314996310074167951142953825183212757110595703125;-0.90960583316531684605621421724208630621433258056640625;0.963051059572882284243178219185210764408111572265625;-0.8817473063929757159939981647767126560211181640625;0.7935564689902567803159172399318777024745941162109375]
      mask Display: e = 0.06;c1 = [120 150 230]/255;c2 = ([120 150 230]+0)/383;c3 = ([120 150 230]+128)/383;patch([0 1 1 0],[0 0 1 1],c1);patch([0 1 1 1-e 1-e 0+e],[0 0 1 1-e 0+e 0+e],c2);patch([0 0 1 1-e 0+e 0+e],[0 1 1 1-e 1-e 0+e],c3);plot([0 1 1 0 0],[0 0 1 1 0]);disp('Weights');
  "IW{1,1}(90,:)'" : Constant  Value=[1.051431316117248826458308030851185321807861328125;-0.54398798558267025260448690460179932415485382080078125;0.1403758236154992733446533748065121471881866455078125;0.94853165771570335795814798984793014824390411376953125;-0.384989371489417531169152653092169202864170074462890625;1.285026930359288943606088650994934141635894775390625;-0.8791103373505995133285750853247009217739105224609375;-0.43548914675894956349821995900128968060016632080078125;0.022662512399713084787489236759938648901879787445068359375;-0.290035038053061022811363045548205263912677764892578125]
      mask Display: e = 0.06;c1 = [120 150 230]/255;c2 = ([120 150 230]+0)/383;c3 = ([120 150 230]+128)/383;patch([0 1 1 0],[0 0 1 1],c1);patch([0 1 1 1-e 1-e 0+e],[0 0 1 1-e 0+e 0+e],c2);patch([0 0 1 1-e 0+e 0+e],[0 1 1 1-e 1-e 0+e],c3);plot([0 1 1 0 0],[0 0 1 1 0]);disp('Weights');
  "IW{1,1}(91,:)'" : Constant  Value=[0.59953840310196915286411467604921199381351470947265625;0.11158827236751349409882294594353879801928997039794921875;-0.442614860281409228104365638500894419848918914794921875;-0.7701134472515420714699985182960517704486846923828125;0.63044069151314496846083557102247141301631927490234375;-0.347849316646802020347450934423250146210193634033203125;-1.025872694946616814348772095399908721446990966796875;-0.5249656038006531577622126860660500824451446533203125;1.0750330293450087726370156815391965210437774658203125;-0.7247125864885795021308467767084948718547821044921875]
      mask Display: e = 0.06;c1 = [120 150 230]/255;c2 = ([120 150 230]+0)/383;c3 = ([120 150 230]+128)/383;patch([0 1 1 0],[0 0 1 1],c1);patch([0 1 1 1-e 1-e 0+e],[0 0 1 1-e 0+e 0+e],c2);patch([0 0 1 1-e 0+e 0+e],[0 1 1 1-e 1-e 0+e],c3);plot([0 1 1 0 0],[0 0 1 1 0]);disp('Weights');
  "IW{1,1}(92,:)'" : Constant  Value=[0.66430495222733565441330938483588397502899169921875;-0.237494067232162542335771604484762065112590789794921875;-1.4058758595996023732510593617917038500308990478515625;-0.587083026582440492546766108716838061809539794921875;-0.411856766996918921552861547752399928867816925048828125;0.1806771229946091128493179667202639393508434295654296875;-0.2182030075757307174821875150882988236844539642333984375;-0.59033076362675751536102097816183231770992279052734375;-0.5422037436892612749517184056458063423633575439453125;-0.327234170999769258258993431809358298778533935546875]
      mask Display: e = 0.06;c1 = [120 150 230]/255;c2 = ([120 150 230]+0)/383;c3 = ([120 150 230]+128)/383;patch([0 1 1 0],[0 0 1 1],c1);patch([0 1 1 1-e 1-e 0+e],[0 0 1 1-e 0+e 0+e],c2);patch([0 0 1 1-e 0+e 0+e],[0 1 1 1-e 1-e 0+e],c3);plot([0 1 1 0 0],[0 0 1 1 0]);disp('Weights');
  "IW{1,1}(93,:)'" : Constant  Value=[-0.3302631584206390247260287651442922651767730712890625;0.0852458510428613092102523296489380300045013427734375;-0.060424136820257497160202575514631462283432483673095703125;0.85860321352863822053080866680829785764217376708984375;-1.07898987574617155615896990639157593250274658203125;0.7630577954628796621960873380885459482669830322265625;0.11899696241098024762639084883630857802927494049072265625;0.90700928791913371096455875886022113263607025146484375;0.97803485095824072015346928310464136302471160888671875;0.69539149528391763777079859210061840713024139404296875]
      mask Display: e = 0.06;c1 = [120 150 230]/255;c2 = ([120 150 230]+0)/383;c3 = ([120 150 230]+128)/383;patch([0 1 1 0],[0 0 1 1],c1);patch([0 1 1 1-e 1-e 0+e],[0 0 1 1-e 0+e 0+e],c2);patch([0 0 1 1-e 0+e 0+e],[0 1 1 1-e 1-e 0+e],c3);plot([0 1 1 0 0],[0 0 1 1 0]);disp('Weights');
  "IW{1,1}(94,:)'" : Constant  Value=[1.186018443418392909194380990811623632907867431640625;0.563330580568514260875190302613191306591033935546875;-0.61707172823085676416354772300110198557376861572265625;0.1921499374536595750040390839785686694085597991943359375;0.54906562756254395640809207179700024425983428955078125;-0.84305040528995067727890955211478285491466522216796875;0.2202868442650489366751997977189603261649608612060546875;1.0492470030332297081798742510727606713771820068359375;0.48523527936053600928545392889645881950855255126953125;0.3630900609934253342458987390273250639438629150390625]
      mask Display: e = 0.06;c1 = [120 150 230]/255;c2 = ([120 150 230]+0)/383;c3 = ([120 150 230]+128)/383;patch([0 1 1 0],[0 0 1 1],c1);patch([0 1 1 1-e 1-e 0+e],[0 0 1 1-e 0+e 0+e],c2);patch([0 0 1 1-e 0+e 0+e],[0 1 1 1-e 1-e 0+e],c3);plot([0 1 1 0 0],[0 0 1 1 0]);disp('Weights');
  "IW{1,1}(95,:)'" : Constant  Value=[0.0776871279191906627392683049038168974220752716064453125;0.62330140950165624502687933272682130336761474609375;-0.116390522855656708411942190650734119117259979248046875;-0.50213933935570154165617395847220905125141143798828125;-0.209509071780552502684003002286772243678569793701171875;-0.792729951579541403106077268603257834911346435546875;1.01573956239322082950593539862893521785736083984375;1.0497991003621940375722942917491309344768524169921875;0.99951601361607222973049147185520268976688385009765625;0.29300321733669243418063388162408955395221710205078125]
      mask Display: e = 0.06;c1 = [120 150 230]/255;c2 = ([120 150 230]+0)/383;c3 = ([120 150 230]+128)/383;patch([0 1 1 0],[0 0 1 1],c1);patch([0 1 1 1-e 1-e 0+e],[0 0 1 1-e 0+e 0+e],c2);patch([0 0 1 1-e 0+e 0+e],[0 1 1 1-e 1-e 0+e],c3);plot([0 1 1 0 0],[0 0 1 1 0]);disp('Weights');
  "IW{1,1}(96,:)'" : Constant  Value=[0.54172006227253721721837109726038761436939239501953125;0.90481494331382972262645125738345086574554443359375;0.372764885683212809919240271483431570231914520263671875;-1.092502070208833497844125304254703223705291748046875;0.4222676449769535711453727344633080065250396728515625;-0.362912959026941372986385658805374987423419952392578125;0.4982691942430015341614080170984379947185516357421875;0.1260224389912012188386114530658232979476451873779296875;-0.652719346263939570462753181345760822296142578125;-1.2438868050972595735714776310487650334835052490234375]
      mask Display: e = 0.06;c1 = [120 150 230]/255;c2 = ([120 150 230]+0)/383;c3 = ([120 150 230]+128)/383;patch([0 1 1 0],[0 0 1 1],c1);patch([0 1 1 1-e 1-e 0+e],[0 0 1 1-e 0+e 0+e],c2);patch([0 0 1 1-e 0+e 0+e],[0 1 1 1-e 1-e 0+e],c3);plot([0 1 1 0 0],[0 0 1 1 0]);disp('Weights');
  "IW{1,1}(97,:)'" : Constant  Value=[-0.13712133349968969042720345896668732166290283203125;-0.67902490976866169969383690840913914144039154052734375;-0.29156901598179041368297248482122085988521575927734375;-1.09199653036838295605548410094343125820159912109375;1.0214003202172692308380419490276835858821868896484375;-0.83339488436484499001011272412142716348171234130859375;0.6853401587047927012719128470052964985370635986328125;-1.0496056032979463878973547252826392650604248046875;-0.04851185808286782863429920098496950231492519378662109375;0.6209703128574091124391998164355754852294921875]
      mask Display: e = 0.06;c1 = [120 150 230]/255;c2 = ([120 150 230]+0)/383;c3 = ([120 150 230]+128)/383;patch([0 1 1 0],[0 0 1 1],c1);patch([0 1 1 1-e 1-e 0+e],[0 0 1 1-e 0+e 0+e],c2);patch([0 0 1 1-e 0+e 0+e],[0 1 1 1-e 1-e 0+e],c3);plot([0 1 1 0 0],[0 0 1 1 0]);disp('Weights');
  "IW{1,1}(98,:)'" : Constant  Value=[0.9810732558117718493662096079788170754909515380859375;0.9522540949847020375074180265073664486408233642578125;0.54827619083491552220976927856099791824817657470703125;-0.924514765178311659354903895291499793529510498046875;0.109319906887178797116888517848565243184566497802734375;0.63469484787636532008292533646454103291034698486328125;0.10222700579901917994352089635867741890251636505126953125;-0.0841202186936103324388369628650252707302570343017578125;-0.360674773197033060601057741223485209047794342041015625;-1.170217351760687751749401286360807716846466064453125]
      mask Display: e = 0.06;c1 = [120 150 230]/255;c2 = ([120 150 230]+0)/383;c3 = ([120 150 230]+128)/383;patch([0 1 1 0],[0 0 1 1],c1);patch([0 1 1 1-e 1-e 0+e],[0 0 1 1-e 0+e 0+e],c2);patch([0 0 1 1-e 0+e 0+e],[0 1 1 1-e 1-e 0+e],c3);plot([0 1 1 0 0],[0 0 1 1 0]);disp('Weights');
  "IW{1,1}(99,:)'" : Constant  Value=[0.80502138240718423833897077201982028782367706298828125;0.1566711219577494318411226004172931425273418426513671875;0.249196748241903798248841894746874459087848663330078125;-0.056686129377532527839900211574786226265132427215576171875;-0.3219565822499748097840210903086699545383453369140625;0.76837497266936816142646193839027546346187591552734375;-1.3039214264229219697455164350685663521289825439453125;-1.2133062219354842081742162918089888989925384521484375;-0.3540594459873369626023986711516045033931732177734375;-0.68255450131037509464704271522350609302520751953125]
      mask Display: e = 0.06;c1 = [120 150 230]/255;c2 = ([120 150 230]+0)/383;c3 = ([120 150 230]+128)/383;patch([0 1 1 0],[0 0 1 1],c1);patch([0 1 1 1-e 1-e 0+e],[0 0 1 1-e 0+e 0+e],c2);patch([0 0 1 1-e 0+e 0+e],[0 1 1 1-e 1-e 0+e],c3);plot([0 1 1 0 0],[0 0 1 1 0]);disp('Weights');
  Mux : Mux  Inputs=100
      mask Display: e = 0.06;c1 = [120 150 230]/255;c2 = ([120 150 230]+0)/383;c3 = ([120 150 230]+128)/383;patch([0 1 1 0],[0 0 1 1],c1);patch([0 1 1 1-e 1-e 0+e],[0 0 1 1-e 0+e 0+e],c2);patch([0 0 1 1-e 0+e 0+e],[0 1 1 1-e 1-e 0+e],c3);plot([0 1 1 0 0],[0 0 1 1 0]);disp('Mux');
  dotprod{1..100} (100 alike) : neural/Weight Functions/dotprod
  "iz{1,1}" : Outport
      mask Display: e = 0.06;c1 = [120 230 180]/255;c2 = ([120 230 180]+0)/(256+128);c3 = ([120 230 180]+128)/(256+128);patch([0 1 1 0],[0 0 1 1],c1);patch([0 1 1 1-e 1-e 0+e],[0 0 1 1-e 0+e 0+e],c2);patch([0 0 1 1-e 0+e 0+e],[0 1 1 1-e 1-e 0+e],c3);plot([0 1 1 0 0],[0 0 1 1 0]);
  wires:
  "IW{1,1}(1,:)'"/1 -> dotprod1/1
  "pd{1,1}"/1 -> dotprod1/2, dotprod2/2, dotprod3/2, dotprod4/2, dotprod5/2, dotprod6/2, dotprod7/2, dotprod8/2, dotprod9/2, dotprod10/2, dotprod11/2, dotprod12/2, dotprod13/2, dotprod14/2, dotprod15/2, dotprod16/2, dotprod17/2, dotprod18/2, dotprod19/2, dotprod20/2, dotprod21/2, dotprod22/2, dotprod23/2, dotprod24/2, dotprod25/2, dotprod26/2, dotprod27/2, dotprod28/2, dotprod29/2, dotprod30/2, dotprod31/2, dotprod32/2, dotprod33/2, dotprod34/2, dotprod35/2, dotprod36/2, dotprod37/2, dotprod38/2, dotprod39/2, dotprod40/2, dotprod41/2, dotprod42/2, dotprod43/2, dotprod44/2, dotprod45/2, dotprod46/2, dotprod47/2, dotprod48/2, dotprod49/2, dotprod50/2, dotprod51/2, dotprod52/2, dotprod53/2, dotprod54/2, dotprod55/2, dotprod56/2, dotprod57/2, dotprod58/2, dotprod59/2, dotprod60/2, dotprod61/2, dotprod62/2, dotprod63/2, dotprod64/2, dotprod65/2, dotprod66/2, dotprod67/2, dotprod68/2, dotprod69/2, dotprod70/2, dotprod71/2, dotprod72/2, dotprod73/2, dotprod74/2, dotprod75/2, dotprod76/2, dotprod77/2, dotprod78/2, dotprod79/2, dotprod80/2, dotprod81/2, dotprod82/2, dotprod83/2, dotprod84/2, dotprod85/2, dotprod86/2, dotprod87/2, dotprod88/2, dotprod89/2, dotprod90/2, dotprod91/2, dotprod92/2, dotprod93/2, dotprod94/2, dotprod95/2, dotprod96/2, dotprod97/2, dotprod98/2, dotprod99/2, dotprod100/2
  dotprod1/1 -> Mux/1
  "IW{1,1}(2,:)'"/1 -> dotprod2/1
  dotprod2/1 -> Mux/2
  "IW{1,1}(3,:)'"/1 -> dotprod3/1
  dotprod3/1 -> Mux/3
  "IW{1,1}(4,:)'"/1 -> dotprod4/1
  dotprod4/1 -> Mux/4
  "IW{1,1}(5,:)'"/1 -> dotprod5/1
  dotprod5/1 -> Mux/5
  "IW{1,1}(6,:)'"/1 -> dotprod6/1
  dotprod6/1 -> Mux/6
  "IW{1,1}(7,:)'"/1 -> dotprod7/1
  dotprod7/1 -> Mux/7
  "IW{1,1}(8,:)'"/1 -> dotprod8/1
  dotprod8/1 -> Mux/8
  "IW{1,1}(9,:)'"/1 -> dotprod9/1
  dotprod9/1 -> Mux/9
  "IW{1,1}(10,:)'"/1 -> dotprod10/1
  dotprod10/1 -> Mux/10
  "IW{1,1}(11,:)'"/1 -> dotprod11/1
  dotprod11/1 -> Mux/11
  "IW{1,1}(12,:)'"/1 -> dotprod12/1
  dotprod12/1 -> Mux/12
  "IW{1,1}(13,:)'"/1 -> dotprod13/1
  dotprod13/1 -> Mux/13
  "IW{1,1}(14,:)'"/1 -> dotprod14/1
  dotprod14/1 -> Mux/14
  "IW{1,1}(15,:)'"/1 -> dotprod15/1
  dotprod15/1 -> Mux/15
  "IW{1,1}(16,:)'"/1 -> dotprod16/1
  dotprod16/1 -> Mux/16
  "IW{1,1}(17,:)'"/1 -> dotprod17/1
  dotprod17/1 -> Mux/17
  "IW{1,1}(18,:)'"/1 -> dotprod18/1
  dotprod18/1 -> Mux/18
  "IW{1,1}(19,:)'"/1 -> dotprod19/1
  dotprod19/1 -> Mux/19
  "IW{1,1}(20,:)'"/1 -> dotprod20/1
  dotprod20/1 -> Mux/20
  "IW{1,1}(21,:)'"/1 -> dotprod21/1
  dotprod21/1 -> Mux/21
  "IW{1,1}(22,:)'"/1 -> dotprod22/1
  dotprod22/1 -> Mux/22
  "IW{1,1}(23,:)'"/1 -> dotprod23/1
  dotprod23/1 -> Mux/23
  "IW{1,1}(24,:)'"/1 -> dotprod24/1
  dotprod24/1 -> Mux/24
  "IW{1,1}(25,:)'"/1 -> dotprod25/1
  dotprod25/1 -> Mux/25
  "IW{1,1}(26,:)'"/1 -> dotprod26/1
  dotprod26/1 -> Mux/26
  "IW{1,1}(27,:)'"/1 -> dotprod27/1
  dotprod27/1 -> Mux/27
  "IW{1,1}(28,:)'"/1 -> dotprod28/1
  dotprod28/1 -> Mux/28
  "IW{1,1}(29,:)'"/1 -> dotprod29/1
  dotprod29/1 -> Mux/29
  "IW{1,1}(30,:)'"/1 -> dotprod30/1
  dotprod30/1 -> Mux/30
  "IW{1,1}(31,:)'"/1 -> dotprod31/1
  dotprod31/1 -> Mux/31
  "IW{1,1}(32,:)'"/1 -> dotprod32/1
  dotprod32/1 -> Mux/32
  "IW{1,1}(33,:)'"/1 -> dotprod33/1
  dotprod33/1 -> Mux/33
  "IW{1,1}(34,:)'"/1 -> dotprod34/1
  dotprod34/1 -> Mux/34
  "IW{1,1}(35,:)'"/1 -> dotprod35/1
  dotprod35/1 -> Mux/35
  "IW{1,1}(36,:)'"/1 -> dotprod36/1
  dotprod36/1 -> Mux/36
  "IW{1,1}(37,:)'"/1 -> dotprod37/1
  dotprod37/1 -> Mux/37
  "IW{1,1}(38,:)'"/1 -> dotprod38/1
  dotprod38/1 -> Mux/38
  "IW{1,1}(39,:)'"/1 -> dotprod39/1
  dotprod39/1 -> Mux/39
  "IW{1,1}(40,:)'"/1 -> dotprod40/1
  dotprod40/1 -> Mux/40
  "IW{1,1}(41,:)'"/1 -> dotprod41/1
  dotprod41/1 -> Mux/41
  "IW{1,1}(42,:)'"/1 -> dotprod42/1
  dotprod42/1 -> Mux/42
  "IW{1,1}(43,:)'"/1 -> dotprod43/1
  dotprod43/1 -> Mux/43
  "IW{1,1}(44,:)'"/1 -> dotprod44/1
  dotprod44/1 -> Mux/44
  "IW{1,1}(45,:)'"/1 -> dotprod45/1
  dotprod45/1 -> Mux/45
  "IW{1,1}(46,:)'"/1 -> dotprod46/1
  dotprod46/1 -> Mux/46
  "IW{1,1}(47,:)'"/1 -> dotprod47/1
  dotprod47/1 -> Mux/47
  "IW{1,1}(48,:)'"/1 -> dotprod48/1
  dotprod48/1 -> Mux/48
  "IW{1,1}(49,:)'"/1 -> dotprod49/1
  dotprod49/1 -> Mux/49
  "IW{1,1}(50,:)'"/1 -> dotprod50/1
  dotprod50/1 -> Mux/50
  "IW{1,1}(51,:)'"/1 -> dotprod51/1
  dotprod51/1 -> Mux/51
  "IW{1,1}(52,:)'"/1 -> dotprod52/1
  dotprod52/1 -> Mux/52
  "IW{1,1}(53,:)'"/1 -> dotprod53/1
  dotprod53/1 -> Mux/53
  "IW{1,1}(54,:)'"/1 -> dotprod54/1
  dotprod54/1 -> Mux/54
  "IW{1,1}(55,:)'"/1 -> dotprod55/1
  dotprod55/1 -> Mux/55
  "IW{1,1}(56,:)'"/1 -> dotprod56/1
  dotprod56/1 -> Mux/56
  "IW{1,1}(57,:)'"/1 -> dotprod57/1
  dotprod57/1 -> Mux/57
  "IW{1,1}(58,:)'"/1 -> dotprod58/1
  dotprod58/1 -> Mux/58
  "IW{1,1}(59,:)'"/1 -> dotprod59/1
  dotprod59/1 -> Mux/59
  "IW{1,1}(60,:)'"/1 -> dotprod60/1
  dotprod60/1 -> Mux/60
  "IW{1,1}(61,:)'"/1 -> dotprod61/1
  dotprod61/1 -> Mux/61
  "IW{1,1}(62,:)'"/1 -> dotprod62/1
  dotprod62/1 -> Mux/62
  "IW{1,1}(63,:)'"/1 -> dotprod63/1
  dotprod63/1 -> Mux/63
  "IW{1,1}(64,:)'"/1 -> dotprod64/1
  dotprod64/1 -> Mux/64
  "IW{1,1}(65,:)'"/1 -> dotprod65/1
  dotprod65/1 -> Mux/65
  "IW{1,1}(66,:)'"/1 -> dotprod66/1
  dotprod66/1 -> Mux/66
  "IW{1,1}(67,:)'"/1 -> dotprod67/1
  dotprod67/1 -> Mux/67
  "IW{1,1}(68,:)'"/1 -> dotprod68/1
  dotprod68/1 -> Mux/68
  "IW{1,1}(69,:)'"/1 -> dotprod69/1
  dotprod69/1 -> Mux/69
  "IW{1,1}(70,:)'"/1 -> dotprod70/1
  dotprod70/1 -> Mux/70
  "IW{1,1}(71,:)'"/1 -> dotprod71/1
  dotprod71/1 -> Mux/71
  "IW{1,1}(72,:)'"/1 -> dotprod72/1
  dotprod72/1 -> Mux/72
  "IW{1,1}(73,:)'"/1 -> dotprod73/1
  dotprod73/1 -> Mux/73
  "IW{1,1}(74,:)'"/1 -> dotprod74/1
  dotprod74/1 -> Mux/74
  "IW{1,1}(75,:)'"/1 -> dotprod75/1
  dotprod75/1 -> Mux/75
  "IW{1,1}(76,:)'"/1 -> dotprod76/1
  dotprod76/1 -> Mux/76
  "IW{1,1}(77,:)'"/1 -> dotprod77/1
  dotprod77/1 -> Mux/77
  "IW{1,1}(78,:)'"/1 -> dotprod78/1
  dotprod78/1 -> Mux/78
  "IW{1,1}(79,:)'"/1 -> dotprod79/1
  dotprod79/1 -> Mux/79
  "IW{1,1}(80,:)'"/1 -> dotprod80/1
  dotprod80/1 -> Mux/80
  "IW{1,1}(81,:)'"/1 -> dotprod81/1
  dotprod81/1 -> Mux/81
  "IW{1,1}(82,:)'"/1 -> dotprod82/1
  dotprod82/1 -> Mux/82
  "IW{1,1}(83,:)'"/1 -> dotprod83/1
  dotprod83/1 -> Mux/83
  "IW{1,1}(84,:)'"/1 -> dotprod84/1
  dotprod84/1 -> Mux/84
  "IW{1,1}(85,:)'"/1 -> dotprod85/1
  dotprod85/1 -> Mux/85
  "IW{1,1}(86,:)'"/1 -> dotprod86/1
  dotprod86/1 -> Mux/86
  "IW{1,1}(87,:)'"/1 -> dotprod87/1
  dotprod87/1 -> Mux/87
  "IW{1,1}(88,:)'"/1 -> dotprod88/1
  dotprod88/1 -> Mux/88
  "IW{1,1}(89,:)'"/1 -> dotprod89/1
  dotprod89/1 -> Mux/89
  "IW{1,1}(90,:)'"/1 -> dotprod90/1
  dotprod90/1 -> Mux/90
  "IW{1,1}(91,:)'"/1 -> dotprod91/1
  dotprod91/1 -> Mux/91
  "IW{1,1}(92,:)'"/1 -> dotprod92/1
  dotprod92/1 -> Mux/92
  "IW{1,1}(93,:)'"/1 -> dotprod93/1
  dotprod93/1 -> Mux/93
  "IW{1,1}(94,:)'"/1 -> dotprod94/1
  dotprod94/1 -> Mux/94
  "IW{1,1}(95,:)'"/1 -> dotprod95/1
  dotprod95/1 -> Mux/95
  "IW{1,1}(96,:)'"/1 -> dotprod96/1
  dotprod96/1 -> Mux/96
  "IW{1,1}(97,:)'"/1 -> dotprod97/1
  dotprod97/1 -> Mux/97
  "IW{1,1}(98,:)'"/1 -> dotprod98/1
  dotprod98/1 -> Mux/98
  "IW{1,1}(99,:)'"/1 -> dotprod99/1
  dotprod99/1 -> Mux/99
  "IW{1,1}(100,:)'"/1 -> dotprod100/1
  dotprod100/1 -> Mux/100
  Mux/1 -> "iz{1,1}"/1
